simulink model "FullFMS_2026_02_17_V0_3_8"  (R2025b)
settings: Solver=ode23tb  StartTime=0.0  StopTime=inf  MaxStep=0.1  RelTol=1e-2
PreLoadFcn:
  | load("BUS_CONFIG.mat")
libraries: opcualib x8
(part 1 of 4)
settings Model: SimulationMode=accelerator  PacingRate=0.100000  Creator=guilh  LastModifiedBy=vitor
settings SolverCC: ZeroCrossControl=DisableAll

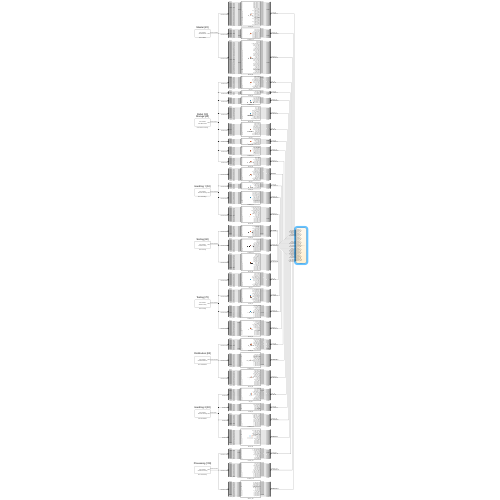
[thumbnail: Simulink's stored preview of the top-level diagram]
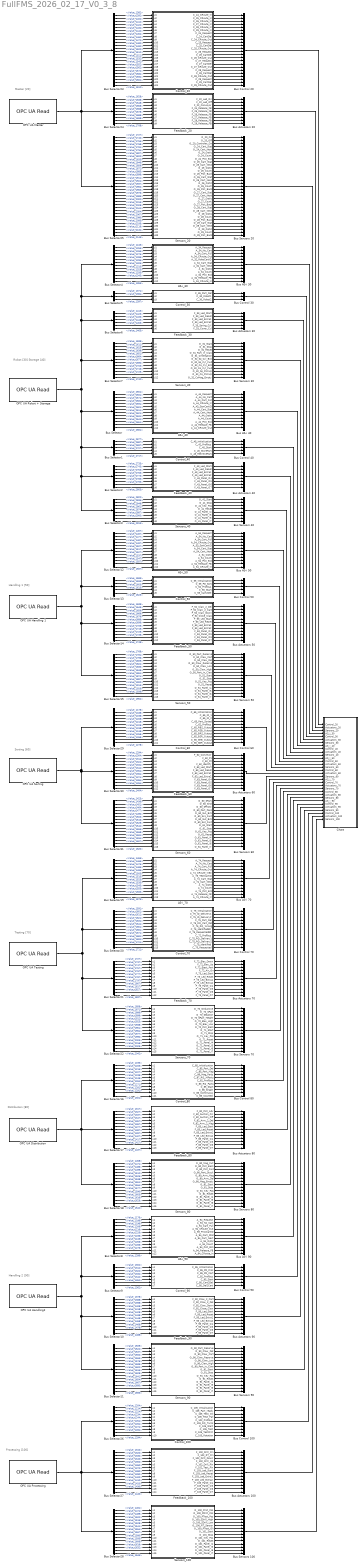
== system FullFMS_2026_02_17_V0_3_8 ==
  note: Master [20]
  note: Robot [30]
      | Storage [40]
  note: Handling 1 [50]
  note: Sorting [60]
  note: Testing [70]
  note: Distribution [80]
  note: Handling 2 [90]
  note: Processing [100]
  AS-i_30 : MATLAB Function  Tag=AS-i  TreatAsAtomicUnit=on
  AS-i_40 : MATLAB Function  TreatAsAtomicUnit=on
  AS-i_50 : MATLAB Function  TreatAsAtomicUnit=on
  AS-i_70 : MATLAB Function  Tag=AS-i  TreatAsAtomicUnit=on
  AS-i_90 : MATLAB Function  Tag=AS-i  TreatAsAtomicUnit=on
  Bus Selector : BusSelector  OutputSignals=Value_2551,Value_2561,Value_2571,Value_2581,Value_2591,Value_2601,Value_2611,Value_2621,Value_2631,Value_2641,Value_2651,Value_2661
  Bus Selector1 : BusSelector  OutputSignals=Value_2677,Value_2687,Value_2697,Value_2707,Value_2717
  Bus Selector10 : BusSelector  OutputSignals=Value_1378,Value_1388,Value_1398,Value_1408,Value_1418,Value_1428,Value_1438,Value_1448,Value_1458,Value_1468,Value_1478,Value_1488
  Bus Selector11 : BusSelector  OutputSignals=Value_1509,Value_1522,Value_1537,Value_1550,Value_1563,Value_1576,Value_1589,Value_1602,Value_1615,Value_1628,Value_1641,Value_1654,Value_1667,Value_1680,Value_1693
  Bus Selector12 : BusSelector  OutputSignals=Value_1457,Value_1467,Value_1477,Value_1487,Value_1497,Value_1507,Value_1517,Value_1527,Value_1537,Value_1547,Value_1557,Value_1567
  Bus Selector13 : BusSelector  OutputSignals=Value_1583,Value_1593,Value_1603,Value_1613,Value_1623
  Bus Selector14 : BusSelector  OutputSignals=Value_1639,Value_1649,Value_1659,Value_1669,Value_1679,Value_1689,Value_1699,Value_1709,Value_1719,Value_1729,Value_1739,Value_1749
  Bus Selector15 : BusSelector  OutputSignals=Value_1768,Value_1781,Value_1796,Value_1809,Value_1822,Value_1835,Value_1848,Value_1861,Value_1874,Value_1887,Value_1900,Value_1913,Value_1926,Value_1939,Value_1952
  Bus Selector16 : BusSelector  OutputSignals=Value_1195,Value_1205,Value_1215,Value_1227,Value_1239,Value_1249,Value_1261,Value_1271,Value_1281,Value_1291,Value_1301
  Bus Selector17 : BusSelector  OutputSignals=Value_1317,Value_1327,Value_1337,Value_1347,Value_1357,Value_1367,Value_1377,Value_1387,Value_1397,Value_1407,Value_1417,Value_1427,Value_1437
  Bus Selector18 : BusSelector  OutputSignals=Value_1458,Value_1471,Value_1486,Value_1499,Value_1512,Value_1525,Value_1538,Value_1551,Value_1564,Value_1577,Value_1590,Value_1603,Value_1616,Value_1629,Value_1642
  Bus Selector19 : BusSelector  OutputSignals=Value_1455,Value_1465,Value_1475,Value_1485,Value_1495,Value_1505,Value_1515,Value_1525,Value_1535,Value_1545,Value_1555,Value_1565,Value_1575
  Bus Selector2 : BusSelector  OutputSignals=Value_2733,Value_2743,Value_2753,Value_2763,Value_2773,Value_2783,Value_2793,Value_2803
  Bus Selector20 : BusSelector  OutputSignals=Value_1591,Value_1601,Value_1611,Value_1621,Value_1631,Value_1641,Value_1651,Value_1661,Value_1671,Value_1681,Value_1691,Value_1701,Value_1711
  Bus Selector21 : BusSelector  OutputSignals=Value_1727,Value_1737,Value_1747,Value_1757,Value_1767,Value_1777,Value_1787,Value_1797,Value_1807,Value_1817,Value_1827,Value_1837
  Bus Selector22 : BusSelector  OutputSignals=Value_1858,Value_1871,Value_1886,Value_1899,Value_1912,Value_1925,Value_1938,Value_1951,Value_1964,Value_1977,Value_1990,Value_2003,Value_2016,Value_2029,Value_2042
  Bus Selector23 : BusSelector  OutputSignals=Value_1382,Value_1392,Value_1402,Value_1412,Value_1422,Value_1432,Value_1442,Value_1452,Value_1462,Value_1472,Value_1482,Value_1492,Value_1502,Value_1512,Value_1522,Value_1532,Value_1542,Value_1552,Value_1562,Value_1572,Value_1582,Value_1592,Value_1602,Value_1612
  Bus Selector24 : BusSelector  OutputSignals=Value_1628,Value_1638,Value_1648,Value_1658,Value_1668,Value_1678,Value_1688,Value_1698,Value_1708
  Bus Selector25 : BusSelector  OutputSignals=Value_1727,Value_1740,Value_1755,Value_1768,Value_1781,Value_1794,Value_1807,Value_1820,Value_1833,Value_1846,Value_1859,Value_1872,Value_1885,Value_1898,Value_1911,Value_1924,Value_1937,Value_1950,Value_1963,Value_1976,Value_1989,Value_2002,Value_2015,Value_2028,Value_2041,Value_2054,Value_2067,Value_2080,Value_2093,Value_2106,Value_2119,Value_2132,Value_2145
  Bus Selector26 : BusSelector  OutputSignals=Value_1204,Value_1214,Value_1224,Value_1234,Value_1244,Value_1254,Value_1264,Value_1274,Value_1284,Value_1294
  Bus Selector27 : BusSelector  OutputSignals=Value_1310,Value_1320,Value_1330,Value_1340,Value_1350,Value_1360,Value_1370,Value_1380,Value_1390,Value_1400,Value_1410,Value_1420,Value_1430,Value_1440
  Bus Selector28 : BusSelector  OutputSignals=Value_1461,Value_1474,Value_1489,Value_1502,Value_1515,Value_1528,Value_1541,Value_1554,Value_1567,Value_1580,Value_1593,Value_1606,Value_1619,Value_1632,Value_1645
  Bus Selector29 : BusSelector  OutputSignals=Value_1178,Value_1188,Value_1198,Value_1208,Value_1218,Value_1228,Value_1238,Value_1248,Value_1258,Value_1268,Value_1278
  Bus Selector3 : BusSelector  OutputSignals=Value_2822,Value_2835,Value_2848,Value_2861,Value_2874,Value_2887,Value_2900,Value_2913
  Bus Selector30 : BusSelector  OutputSignals=Value_1294,Value_1304,Value_1314,Value_1324,Value_1334,Value_1344,Value_1354,Value_1364,Value_1374,Value_1384,Value_1394,Value_1404
  Bus Selector31 : BusSelector  OutputSignals=Value_1423,Value_1436,Value_1451,Value_1464,Value_1477,Value_1490,Value_1503,Value_1516,Value_1529,Value_1542,Value_1555,Value_1568,Value_1581,Value_1594,Value_1607,Value_1620
  Bus Selector4 : BusSelector  OutputSignals=Value_1245,Value_1255,Value_1265,Value_1275,Value_1285,Value_1295,Value_1305,Value_1315,Value_1325,Value_1335,Value_1345,Value_1355
  Bus Selector5 : BusSelector  OutputSignals=Value_1371,Value_1384,Value_1397
  Bus Selector6 : BusSelector  OutputSignals=Value_1413,Value_1423,Value_1433,Value_1443,Value_1453,Value_1463
  Bus Selector7 : BusSelector  OutputSignals=Value_1599,Value_1612,Value_1625,Value_1638,Value_1651,Value_1664,Value_1677,Value_1690,Value_1703,Value_1716,Value_1729,Value_1742
  Bus Selector8 : BusSelector  OutputSignals=Value_1176,Value_1186,Value_1196,Value_1206,Value_1216,Value_1226,Value_1236,Value_1246,Value_1256,Value_1266,Value_1276,Value_1286
  Bus Selector9 : BusSelector  OutputSignals=Value_1302,Value_1312,Value_1322,Value_1332,Value_1342,Value_1352,Value_1362
  Bus AS-i 30 : BusCreator  Inputs=12  OutDataTypeStr=Bus: B_AS_i_30  NonVirtualBus=on
  Bus AS-i 40 : BusCreator  Inputs=12  OutDataTypeStr=Bus: B_AS_i_40  NonVirtualBus=on
  Bus AS-i 50 : BusCreator  Inputs=12  OutDataTypeStr=Bus: B_AS_i_50  NonVirtualBus=on
  Bus AS-i 70 : BusCreator  Inputs=13  OutDataTypeStr=Bus: B_AS_i_70  NonVirtualBus=on
  Bus AS-i 90 : BusCreator  Inputs=12  OutDataTypeStr=Bus: B_AS_i_90  NonVirtualBus=on
  Bus Actuators 100 : BusCreator  Inputs=14  OutDataTypeStr=Bus: B_Actuators_100  NonVirtualBus=on
  Bus Actuators 20 : BusCreator  Inputs=9  OutDataTypeStr=Bus: B_Actuators_20  NonVirtualBus=on
  Bus Actuators 30 : BusCreator  Inputs=6  OutDataTypeStr=Bus: B_Actuators_30  NonVirtualBus=on
  Bus Actuators 40 : BusCreator  Inputs=8  OutDataTypeStr=Bus: B_Actuators_40  NonVirtualBus=on
  Bus Actuators 50 : BusCreator  Inputs=12  OutDataTypeStr=Bus: B_Actuators_50  NonVirtualBus=on
  Bus Actuators 60 : BusCreator  Inputs=12  OutDataTypeStr=Bus: B_Actuators_60  NonVirtualBus=on
  Bus Actuators 70 : BusCreator  Inputs=12  OutDataTypeStr=Bus: B_Actuators_70  NonVirtualBus=on
  Bus Actuators 80 : BusCreator  Inputs=13  OutDataTypeStr=Bus: B_Actuators_80  NonVirtualBus=on
  Bus Actuators 90 : BusCreator  Inputs=12  OutDataTypeStr=Bus: B_Actuators_90  NonVirtualBus=on
  Bus Control 100 : BusCreator  Inputs=10  OutDataTypeStr=Bus: B_Control_100  NonVirtualBus=on
  Bus Control 20 : BusCreator  Inputs=24  OutDataTypeStr=Bus: B_Control_20  NonVirtualBus=on
  Bus Control 30 : BusCreator  Inputs=3  OutDataTypeStr=Bus: B_Control_30  NonVirtualBus=on
  Bus Control 40 : BusCreator  Inputs=5  OutDataTypeStr=Bus: B_Control_40  NonVirtualBus=on
  Bus Control 50 : BusCreator  Inputs=5  OutDataTypeStr=Bus: B_Control_50  NonVirtualBus=on
  Bus Control 60 : BusCreator  Inputs=11  OutDataTypeStr=Bus: B_Control_60  NonVirtualBus=on
  Bus Control 70 : BusCreator  Inputs=13  OutDataTypeStr=Bus: B_Control_70  NonVirtualBus=on
  Bus Control 80 : BusCreator  Inputs=11  OutDataTypeStr=Bus: B_Control_80  NonVirtualBus=on
  Bus Control 90 : BusCreator  Inputs=7  OutDataTypeStr=Bus: B_Control_90  NonVirtualBus=on
  Bus Sensors 100 : BusCreator  Inputs=15  OutDataTypeStr=Bus: B_Sensors_100  NonVirtualBus=on
  Bus Sensors 20 : BusCreator  Inputs=33  OutDataTypeStr=Bus: B_Sensors_20  NonVirtualBus=on
  Bus Sensors 30 : BusCreator  Inputs=12  OutDataTypeStr=Bus: B_Sensors_30  NonVirtualBus=on
  Bus Sensors 40 : BusCreator  Inputs=8  OutDataTypeStr=Bus: B_Sensors_40  NonVirtualBus=on
  Bus Sensors 50 : BusCreator  Inputs=15  OutDataTypeStr=Bus: B_Sensors_50  NonVirtualBus=on
  Bus Sensors 60 : BusCreator  Inputs=16  OutDataTypeStr=Bus: B_Sensors_60  NonVirtualBus=on
  Bus Sensors 70 : BusCreator  Inputs=15  OutDataTypeStr=Bus: B_Sensors_70  NonVirtualBus=on
  Bus Sensors 80 : BusCreator  Inputs=15  OutDataTypeStr=Bus: B_Sensors_80  NonVirtualBus=on
  Bus Sensors 90 : BusCreator  Inputs=15  OutDataTypeStr=Bus: B_Sensors_90  NonVirtualBus=on
  Chart : Stateflow chart  TreatAsAtomicUnit=on
      settings: PortSchema="{\"entries\":[{\"content\":{\"sides\":[{\"content\":{\"connectorIds\":[\"In18\",\"In12\",\"In24\",\"In8\",\"In19\",\"In13\",\"In25\",\"In30\",\"In29\",\"In31\",\"In32\",\"In9\",\"In20\",\"In14\",\"In26\",\"In21\",\"In15\",\"In27\",\"In4\",\"In5\",\"In6\",\"In7\",\"In1\",\"In2\",\"In3\",\"In10\",\"In22\",\"In16\",\"In28\",\"In17\",\"In11\",\"In23\"]},\"type\":\"ConnectorPlacement.EquallySpacedRectSide\",\"uuid\":\"e54bf7d4-7c7d-41d9-a8b8-f479ac319a99\"},{\"content\":{\"side\":\"RIGHT\"},\"type\":\"ConnectorPlacement.EquallySpacedRectSide\",\"uuid\":\"d3c20706-71bd-4e26-b40f-0ee7e71b06ee\"},{\"content\":{\"side\":\"TOP\"},\"type\":\"ConnectorPlacement.EquallySpacedRectSide\",\"uuid\":\"ecfb6920-e95b-4ed8-99f9-df5ce878328e\"}]},\"type\":\"ConnectorPlacement.EquallySpacedConnector\",\"uuid\":\"2e714192-4eea-4e1a-8945-7c827feed48f\"}],\"packageUris\":[\"http://schema.mathworks.com/mf0/Connector/R2020b\"],\"version\":\"1.0\"}"
  Control_100 : MATLAB Function  Tag=Control  TreatAsAtomicUnit=on
  Control_20 : MATLAB Function  Tag=Control  TreatAsAtomicUnit=on
  Control_30 : MATLAB Function  Tag=Control  TreatAsAtomicUnit=on
  Control_40 : MATLAB Function  TreatAsAtomicUnit=on
  Control_50 : MATLAB Function  TreatAsAtomicUnit=on
  Control_60 : MATLAB Function  Tag=Control  TreatAsAtomicUnit=on
  Control_70 : MATLAB Function  Tag=Control  TreatAsAtomicUnit=on
  Control_80 : MATLAB Function  Tag=Control  TreatAsAtomicUnit=on
  Control_90 : MATLAB Function  Tag=Control  TreatAsAtomicUnit=on
  Feedback_100 : MATLAB Function  Tag=Actuators  TreatAsAtomicUnit=on
  Feedback_20 : MATLAB Function  Tag=Actuators  TreatAsAtomicUnit=on
  Feedback_30 : MATLAB Function  Tag=Actuators  TreatAsAtomicUnit=on
  Feedback_40 : MATLAB Function  TreatAsAtomicUnit=on
  Feedback_50 : MATLAB Function  TreatAsAtomicUnit=on
  Feedback_60 : MATLAB Function  Tag=Actuators  TreatAsAtomicUnit=on
  Feedback_70 : MATLAB Function  Tag=Actuators  TreatAsAtomicUnit=on
  Feedback_80 : MATLAB Function  Tag=Actuators  TreatAsAtomicUnit=on
  Feedback_90 : MATLAB Function  Tag=Actuators  TreatAsAtomicUnit=on
  OPC UA Distribution : opcualib/OPC UA Read  SelectedServer=AAS OPC Distribution  ServerList=AAS OPC Distribution  NodeList={ '1', 'Value', '6', '1195', '1'; '2', 'Value', '6', '1205', '1'; '3', 'Value', '6', '1215', '1'; '4', 'Value', '6', '1227', '1'; '5', 'Value', '6', '1239', '1'; '6', 'Value', '6', '1249', '1'; '7', 'Value', '6', '1261', '1'; '8', 'Value', '6', '1271', '1'; '9', 'Value', '6', '1281', '1'; '10', 'Value', '6', '1291', '1'; '11', 'Value', '6', '1301', '1'; '12', 'Value', '6', '1317', '1'; '13', 'Value', '6', '1327', '1'; '14', 'Value', '6', '1337', '1'; '15', 'Value', '6', '1347', '1'; '16', 'Value', '6', '1357', '1'; '17', 'Value', '6', '1367', '1'; '18', 'Value', '6', '1377', '1'; '19', 'Value', '6', '1387', '1'; '20', 'Value', '6', '1397', '1'; '21', 'Value', '6', '1407', '1'; '22', 'Value', '6', '1417', '1'; '23', 'Value', '6', '1427', '1'; '24', 'Value', '6', '1437', '1'; '25', 'Value', '6', '1458', '1'; '26', 'Value', '6', '1471', '1'; '27', 'Value', '6', '1486', '1'; '28', 'Value', '6', '1499', '1'; '29', 'Value', '6', '1512', '1'; '30', 'Value', '6', '1525', '1'; '31', 'Value', '6', '1538', '1'; '32', 'Value', '6', '1551', '1'; '33', 'Value', '6', '1564', '1'; '34', 'Value', '6', '1577', '1'; '35', 'Value', '6', '1590', '1'; '36', 'Value', '6', '1603', '1'; '37', 'Value', '6', '1616', '1'; '38', 'Value', '6', '1629', '1'; '39', 'Value', '6', '1642', '1' }  ShowQualityPort=off  ShowTimestampPort=off  ShowTimestampPortAs=Seconds since start  SampleTime=-1
  OPC UA Handling 1 : opcualib/OPC UA Read  SelectedServer=AAS OPC Handling1  ServerList=AAS OPC Handling1  NodeList={ '1', 'Value', '6', '1457', '1'; '2', 'Value', '6', '1467', '1'; '3', 'Value', '6', '1477', '1'; '4', 'Value', '6', '1487', '1'; '5', 'Value', '6', '1497', '1'; '6', 'Value', '6', '1507', '1'; '7', 'Value', '6', '1517', '1'; '8', 'Value', '6', '1527', '1'; '9', 'Value', '6', '1537', '1'; '10', 'Value', '6', '1547', '1'; '11', 'Value', '6', '1557', '1'; '12', 'Value', '6', '1567', '1'; '13', 'Value', '6', '1583', '1'; '14', 'Value', '6', '1593', '1'; '15', 'Value', '6', '1603', '1'; '16', 'Value', '6', '1613', '1'; '17', 'Value', '6', '1623', '1'; '18', 'Value', '6', '1639', '1'; '19', 'Value', '6', '1649', '1'; '20', 'Value', '6', '1659', '1'; '21', 'Value', '6', '1669', '1'; '22', 'Value', '6', '1679', '1'; '23', 'Value', '6', '1689', '1'; '24', 'Value', '6', '1699', '1'; '25', 'Value', '6', '1709', '1'; '26', 'Value', '6', '1719', '1'; '27', 'Value', '6', '1729', '1'; '28', 'Value', '6', '1739', '1'; '29', 'Value', '6', '1749', '1'; '30', 'Value', '6', '1768', '1'; '31', 'Value', '6', '1781', '1'; '32', 'Value', '6', '1796', '1'; '33', 'Value', '6', '1809', '1'; '34', 'Value', '6', '1822', '1'; '35', 'Value', '6', '1835', '1'; '36', 'Value', '6', '1848', '1'; '37', 'Value', '6', '1861', '1'; '38', 'Value', '6', '1874', '1'; '39', 'Value', '6', '1887', '1'; '40', 'Value', '6', '1900', '1'; '41', 'Value', '6', '1913', '1'; '42', 'Value', '6', '1926', '1'; '43', 'Value', '6', '1939', '1'; '44', 'Value', '6', '1952', '1' }  ShowQualityPort=off  ShowTimestampPort=off  ShowTimestampPortAs=Seconds since start  SampleTime=-1
  OPC UA Handling2 : opcualib/OPC UA Read  SelectedServer=AAS OPC Handling2  ServerList=AAS OPC Handling2  NodeList={ '1', 'Value', '6', '1176', '1'; '2', 'Value', '6', '1186', '1'; '3', 'Value', '6', '1196', '1'; '4', 'Value', '6', '1206', '1'; '5', 'Value', '6', '1216', '1'; '6', 'Value', '6', '1226', '1'; '7', 'Value', '6', '1236', '1'; '8', 'Value', '6', '1246', '1'; '9', 'Value', '6', '1256', '1'; '10', 'Value', '6', '1266', '1'; '11', 'Value', '6', '1276', '1'; '12', 'Value', '6', '1286', '1'; '13', 'Value', '6', '1302', '1'; '14', 'Value', '6', '1312', '1'; '15', 'Value', '6', '1322', '1'; '16', 'Value', '6', '1332', '1'; '17', 'Value', '6', '1342', '1'; '18', 'Value', '6', '1352', '1'; '19', 'Value', '6', '1362', '1'; '20', 'Value', '6', '1378', '1'; '21', 'Value', '6', '1388', '1'; '22', 'Value', '6', '1398', '1'; '23', 'Value', '6', '1408', '1'; '24', 'Value', '6', '1418', '1'; '25', 'Value', '6', '1428', '1'; '26', 'Value', '6', '1438', '1'; '27', 'Value', '6', '1448', '1'; '28', 'Value', '6', '1458', '1'; '29', 'Value', '6', '1468', '1'; '30', 'Value', '6', '1478', '1'; '31', 'Value', '6', '1488', '1'; '32', 'Value', '6', '1509', '1'; '33', 'Value', '6', '1522', '1'; '34', 'Value', '6', '1537', '1'; '35', 'Value', '6', '1550', '1'; '36', 'Value', '6', '1563', '1'; '37', 'Value', '6', '1576', '1'; '38', 'Value', '6', '1589', '1'; '39', 'Value', '6', '1602', '1'; '40', 'Value', '6', '1615', '1'; '41', 'Value', '6', '1628', '1'; '42', 'Value', '6', '1641', '1'; '43', 'Value', '6', '1654', '1'; '44', 'Value', '6', '1667', '1'; '45', 'Value', '6', '1680', '1'; '46', 'Value', '6', '1693', '1' }  ShowQualityPort=off  ShowTimestampPort=off  ShowTimestampPortAs=Seconds since start  SampleTime=-1
  OPC UA Master : opcualib/OPC UA Read  SelectedServer=AAS OPC Master  ServerList=AAS OPC Master  NodeList={ '1', 'Value', '6', '1382', '1'; '2', 'Value', '6', '1392', '1'; '3', 'Value', '6', '1402', '1'; '4', 'Value', '6', '1412', '1'; '5', 'Value', '6', '1422', '1'; '6', 'Value', '6', '1432', '1'; '7', 'Value', '6', '1442', '1'; '8', 'Value', '6', '1452', '1'; '9', 'Value', '6', '1462', '1'; '10', 'Value', '6', '1472', '1'; '11', 'Value', '6', '1482', '1'; '12', 'Value', '6', '1492', '1'; '13', 'Value', '6', '1502', '1'; '14', 'Value', '6', '1512', '1'; '15', 'Value', '6', '1522', '1'; '16', 'Value', '6', '1532', '1'; '17', 'Value', '6', '1542', '1'; '18', 'Value', '6', '1552', '1'; '19', 'Value', '6', '1562', '1'; '20', 'Value', '6', '1572', '1'; '21', 'Value', '6', '1582', '1'; '22', 'Value', '6', '1592', '1'; '23', 'Value', '6', '1602', '1'; '24', 'Value', '6', '1612', '1'; '25', 'Value', '6', '1628', '1'; '26', 'Value', '6', '1638', '1'; '27', 'Value', '6', '1648', '1'; '28', 'Value', '6', '1658', '1'; '29', 'Value', '6', '1668', '1'; '30', 'Value', '6', '1678', '1'; '31', 'Value', '6', '1688', '1'; '32', 'Value', '6', '1698', '1'; '33', 'Value', '6', '1708', '1'; '34', 'Value', '6', '1727', '1'; '35', 'Value', '6', '1740', '1'; '36', 'Value', '6', '1755', '1'; '37', 'Value', '6', '1768', '1'; '38', 'Value', '6', '1781', '1'; '39', 'Value', '6', '1794', '1'; '40', 'Value', '6', '1807', '1'; '41', 'Value', '6', '1820', '1'; '42', 'Value', '6', '1833', '1'; '43', 'Value', '6', '1846', '1'; '44', 'Value', '6', '1859', '1'; '45', 'Value', '6', '1872', '1'; '46', 'Value', '6', '1885', '1'; '47', 'Value', '6', '1898', '1'; '48', 'Value', '6', '1911', '1'; '49', 'Value', '6', '1924', '1'; '50', 'Value', '6', '1937', '1'; '51', 'Value', '6', '1950', '1'; '52', 'Value', '6', '1963', '1'; '53', 'Value', '6', '1976', '1'; '54', 'Value', '6', '1989', '1'; '55', 'Value', '6', '2002', '1'; '56', 'Value', '6', '2015', '1'; '57', 'Value', '6', '2028', '1'; '58', 'Value', '6', '2041', '1'; '59', 'Value', '6', '2054', '1'; '60', 'Value', '6', '2067', '1'; '61', 'Value', '6', '2080', '1'; '62', 'Value', '6', '2093', '1'; '63', 'Value', '6', '2106', '1'; '64', 'Value', '6', '2119', '1'; '65', 'Value', '6', '2132', '1'; '66', 'Value', '6', '2145', '1' }  ShowQualityPort=off  ShowTimestampPort=off  ShowTimestampPortAs=Seconds since start  SampleTime=-1
  OPC UA Processing : opcualib/OPC UA Read  SelectedServer=AAS OPC Processing  ServerList=AAS OPC Processing  NodeList={ '1', 'Value', '6', '1204', '1'; '2', 'Value', '6', '1214', '1'; '3', 'Value', '6', '1224', '1'; '4', 'Value', '6', '1234', '1'; '5', 'Value', '6', '1244', '1'; '6', 'Value', '6', '1254', '1'; '7', 'Value', '6', '1264', '1'; '8', 'Value', '6', '1274', '1'; '9', 'Value', '6', '1284', '1'; '10', 'Value', '6', '1294', '1'; '11', 'Value', '6', '1310', '1'; '12', 'Value', '6', '1320', '1'; '13', 'Value', '6', '1330', '1'; '14', 'Value', '6', '1340', '1'; '15', 'Value', '6', '1350', '1'; '16', 'Value', '6', '1360', '1'; '17', 'Value', '6', '1370', '1'; '18', 'Value', '6', '1380', '1'; '19', 'Value', '6', '1390', '1'; '20', 'Value', '6', '1400', '1'; '21', 'Value', '6', '1410', '1'; '22', 'Value', '6', '1420', '1'; '23', 'Value', '6', '1430', '1'; '24', 'Value', '6', '1440', '1'; '25', 'Value', '6', '1461', '1'; '26', 'Value', '6', '1474', '1'; '27', 'Value', '6', '1489', '1'; '28', 'Value', '6', '1502', '1'; '29', 'Value', '6', '1515', '1'; '30', 'Value', '6', '1528', '1'; '31', 'Value', '6', '1541', '1'; '32', 'Value', '6', '1554', '1'; '33', 'Value', '6', '1567', '1'; '34', 'Value', '6', '1580', '1'; '35', 'Value', '6', '1593', '1'; '36', 'Value', '6', '1606', '1'; '37', 'Value', '6', '1619', '1'; '38', 'Value', '6', '1632', '1'; '39', 'Value', '6', '1645', '1' }  ShowQualityPort=off  ShowTimestampPort=off  ShowTimestampPortAs=Seconds since start  SampleTime=-1
  OPC UA Robot + Storage : opcualib/OPC UA Read  SelectedServer=Node-RED OPCUA  ServerList=Node-RED OPCUA  NodeList={ '1', 'Value', '6', '2551', '1'; '2', 'Value', '6', '2561', '1'; '3', 'Value', '6', '2571', '1'; '4', 'Value', '6', '2581', '1'; '5', 'Value', '6', '2591', '1'; '6', 'Value', '6', '2601', '1'; '7', 'Value', '6', '2611', '1'; '8', 'Value', '6', '2621', '1'; '9', 'Value', '6', '2631', '1'; '10', 'Value', '6', '2641', '1'; '11', 'Value', '6', '2651', '1'; '12', 'Value', '6', '2661', '1'; '13', 'Value', '6', '2677', '1'; '14', 'Value', '6', '2687', '1'; '15', 'Value', '6', '2697', '1'; '16', 'Value', '6', '2707', '1'; '17', 'Value', '6', '2717', '1'; '18', 'Value', '6', '2733', '1'; '19', 'Value', '6', '2743', '1'; '20', 'Value', '6', '2753', '1'; '21', 'Value', '6', '2763', '1'; '22', 'Value', '6', '2773', '1'; '23', 'Value', '6', '2783', '1'; '24', 'Value', '6', '2793', '1'; '25', 'Value', '6', '2803', '1'; '26', 'Value', '6', '2822', '1'; '27', 'Value', '6', '2835', '1'; '28', 'Value', '6', '2848', '1'; '29', 'Value', '6', '2861', '1'; '30', 'Value', '6', '2874', '1'; '31', 'Value', '6', '2887', '1'; '32', 'Value', '6', '2900', '1'; '33', 'Value', '6', '2913', '1'; '34', 'Value', '6', '1245', '1'; '35', 'Value', '6', '1255', '1'; '36', 'Value', '6', '1265', '1'; '37', 'Value', '6', '1275', '1'; '38', 'Value', '6', '1285', '1'; '39', 'Value', '6', '1295', '1'; '40', 'Value', '6', '1305', '1'; '41', 'Value', '6', '1315', '1'; '42', 'Value', '6', '1325', '1'; '43', 'Value', '6', '1335', '1'; '44', 'Value', '6', '1345', '1'; '45', 'Value', '6', '1355', '1'; '46', 'Value', '6', '1371', '1'; '47', 'Value', '6', '1384', '1'; '48', 'Value', '6', '1397', '1'; '49', 'Value', '6', '1413', '1'; '50', 'Value', '6', '1423', '1'; '51', 'Value', '6', '1433', '1'; '52', 'Value', '6', '1443', '1'; '53', 'Value', '6', '1453', '1'; '54', 'Value', '6', '1463', '1'; '55', 'Value', '6', '1599', '1'; '56', 'Value', '6', '1612', '1'; '57', 'Value', '6', '1625', '1'; '58', 'Value', '6', '1638', '1'; '59', 'Value', '6', '1651', '1'; '60', 'Value', '6', '1664', '1'; '61', 'Value', '6', '1677', '1'; '62', 'Value', '6', '1690', '1'; '63', 'Value', '6', '1703', '1'; '64', 'Value', '6', '1716', '1'; '65', 'Value', '6', '1729', '1'; '66', 'Value', '6', '1742', '1' }  ShowQualityPort=off  ShowTimestampPort=off  ShowTimestampPortAs=Seconds since start  SampleTime=-1
  OPC UA Sorting : opcualib/OPC UA Read  SelectedServer=AAS OPC Sorting  ServerList=AAS OPC Sorting  NodeList={ '1', 'Value', '6', '1178', '1'; '2', 'Value', '6', '1188', '1'; '3', 'Value', '6', '1198', '1'; '4', 'Value', '6', '1208', '1'; '5', 'Value', '6', '1218', '1'; '6', 'Value', '6', '1228', '1'; '7', 'Value', '6', '1238', '1'; '8', 'Value', '6', '1248', '1'; '9', 'Value', '6', '1258', '1'; '10', 'Value', '6', '1268', '1'; '11', 'Value', '6', '1278', '1'; '12', 'Value', '6', '1294', '1'; '13', 'Value', '6', '1304', '1'; '14', 'Value', '6', '1314', '1'; '15', 'Value', '6', '1324', '1'; '16', 'Value', '6', '1334', '1'; '17', 'Value', '6', '1344', '1'; '18', 'Value', '6', '1354', '1'; '19', 'Value', '6', '1364', '1'; '20', 'Value', '6', '1374', '1'; '21', 'Value', '6', '1384', '1'; '22', 'Value', '6', '1394', '1'; '23', 'Value', '6', '1404', '1'; '24', 'Value', '6', '1423', '1'; '25', 'Value', '6', '1436', '1'; '26', 'Value', '6', '1451', '1'; '27', 'Value', '6', '1464', '1'; '28', 'Value', '6', '1477', '1'; '29', 'Value', '6', '1490', '1'; '30', 'Value', '6', '1503', '1'; '31', 'Value', '6', '1516', '1'; '32', 'Value', '6', '1529', '1'; '33', 'Value', '6', '1542', '1'; '34', 'Value', '6', '1555', '1'; '35', 'Value', '6', '1568', '1'; '36', 'Value', '6', '1581', '1'; '37', 'Value', '6', '1594', '1'; '38', 'Value', '6', '1607', '1'; '39', 'Value', '6', '1620', '1' }  ShowQualityPort=off  ShowTimestampPort=off  ShowTimestampPortAs=Seconds since start  SampleTime=-1
  OPC UA Testing : opcualib/OPC UA Read  SelectedServer=AAS OPC Testing  ServerList=AAS OPC Testing  NodeList={ '1', 'Value', '6', '1455', '1'; '2', 'Value', '6', '1465', '1'; '3', 'Value', '6', '1475', '1'; '4', 'Value', '6', '1485', '1'; '5', 'Value', '6', '1495', '1'; '6', 'Value', '6', '1505', '1'; '7', 'Value', '6', '1515', '1'; '8', 'Value', '6', '1525', '1'; '9', 'Value', '6', '1535', '1'; '10', 'Value', '6', '1545', '1'; '11', 'Value', '6', '1555', '1'; '12', 'Value', '6', '1565', '1'; '13', 'Value', '6', '1575', '1'; '14', 'Value', '6', '1591', '1'; '15', 'Value', '6', '1601', '1'; '16', 'Value', '6', '1611', '1'; '17', 'Value', '6', '1621', '1'; '18', 'Value', '6', '1631', '1'; '19', 'Value', '6', '1641', '1'; '20', 'Value', '6', '1651', '1'; '21', 'Value', '6', '1661', '1'; '22', 'Value', '6', '1671', '1'; '23', 'Value', '6', '1681', '1'; '24', 'Value', '6', '1691', '1'; '25', 'Value', '6', '1701', '1'; '26', 'Value', '6', '1711', '1'; '27', 'Value', '6', '1727', '1'; '28', 'Value', '6', '1737', '1'; '29', 'Value', '6', '1747', '1'; '30', 'Value', '6', '1757', '1'; '31', 'Value', '6', '1767', '1'; '32', 'Value', '6', '1777', '1'; '33', 'Value', '6', '1787', '1'; '34', 'Value', '6', '1797', '1'; '35', 'Value', '6', '1807', '1'; '36', 'Value', '6', '1817', '1'; '37', 'Value', '6', '1827', '1'; '38', 'Value', '6', '1837', '1'; '39', 'Value', '6', '1858', '1'; '40', 'Value', '6', '1871', '1'; '41', 'Value', '6', '1886', '1'; '42', 'Value', '6', '1899', '1'; '43', 'Value', '6', '1912', '1'; '44', 'Value', '6', '1925', '1'; '45', 'Value', '6', '1938', '1'; '46', 'Value', '6', '1951', '1'; '47', 'Value', '6', '1964', '1'; '48', 'Value', '6', '1977', '1'; '49', 'Value', '6', '1990', '1'; '50', 'Value', '6', '2003', '1'; '51', 'Value', '6', '2016', '1'; '52', 'Value', '6', '2029', '1'; '53', 'Value', '6', '2042', '1' }  ShowQualityPort=off  ShowTimestampPort=off  ShowTimestampPortAs=Seconds since start  SampleTime=-1
  Sensors_100 : MATLAB Function  Tag=Sensors  TreatAsAtomicUnit=on
  Sensors_20 : MATLAB Function  Tag=Sensor  TreatAsAtomicUnit=on
  Sensors_30 : MATLAB Function  Tag=Sensors  TreatAsAtomicUnit=on
  Sensors_40 : MATLAB Function  TreatAsAtomicUnit=on
  Sensors_50 : MATLAB Function  Tag=Sensors  TreatAsAtomicUnit=on
  Sensors_60 : MATLAB Function  Tag=Sensors  TreatAsAtomicUnit=on
  Sensors_70 : MATLAB Function  Tag=Sensors  TreatAsAtomicUnit=on
  Sensors_80 : MATLAB Function  Tag=Sensors  TreatAsAtomicUnit=on
  Sensors_90 : MATLAB Function  Tag=Sensors  TreatAsAtomicUnit=on
  wires:
  Feedback_80/1(F_82_Pist_Adv) -> Bus Actuators 80/1
  Feedback_80/2(F_82_Suction_On) -> Bus Actuators 80/2
  Feedback_80/3(F_82_Suction_Off) -> Bus Actuators 80/3
  Feedback_80/4(F_82_Arm_2_Del) -> Bus Actuators 80/4
  Feedback_80/5(F_82_Arm_2_Mag) -> Bus Actuators 80/5
  Feedback_80/6(F_83_Led_Start) -> Bus Actuators 80/6
  Feedback_80/7(F_83_Led_Reset) -> Bus Actuators 80/7
  Feedback_80/8(F_83_Led_Extra1) -> Bus Actuators 80/8
  Feedback_80/9(F_83_Led_Extra2) -> Bus Actuators 80/9
  Feedback_80/10(F_83_Panel_O4) -> Bus Actuators 80/10
  Feedback_80/11(F_83_Panel_O5) -> Bus Actuators 80/11
  Feedback_80/12(F_83_Panel_O6) -> Bus Actuators 80/12
  Feedback_80/13(F_83_Panel_O7) -> Bus Actuators 80/13
  Sensors_80/1(O_80_Mag_Full) -> Bus Sensors 80/1
  Sensors_80/2(O_80_Pist_Back) -> Bus Sensors 80/2
  Sensors_80/3(O_80_Pist_Fwd) -> Bus Sensors 80/3
  Sensors_80/4(O_80_Part_Stuck) -> Bus Sensors 80/4
  Sensors_80/5(O_80_Arm_Mag) -> Bus Sensors 80/5
  Sensors_80/6(O_80_Arm_Del) -> Bus Sensors 80/6
  Sensors_80/7(O_80_Mag_Empty) -> Bus Sensors 80/7
  Sensors_80/8(O_81_Start) -> Bus Sensors 80/8
  Sensors_80/9(O_81_Stop) -> Bus Sensors 80/9
  Sensors_80/10(O_81_Key_Pos) -> Bus Sensors 80/10
  Sensors_80/11(O_81_Reset) -> Bus Sensors 80/11
  Sensors_80/12(O_81_Panel_I4) -> Bus Sensors 80/12
  Sensors_80/13(O_81_Panel_I5) -> Bus Sensors 80/13
  Sensors_80/14(O_81_Panel_I6) -> Bus Sensors 80/14
  Sensors_80/15(O_81_Panel_I7) -> Bus Sensors 80/15
  AS-i_70/1(A_74_Request) -> Bus AS-i 70/1
  AS-i_70/2(A_74_No_Cart) -> Bus AS-i 70/2
  AS-i_70/3(A_74_Cart_Full) -> Bus AS-i 70/3
  AS-i_70/4(A_74_CRoute_Out) -> Bus AS-i 70/4
  AS-i_70/5(A_74_CRoute_In80) -> Bus AS-i 70/5
  AS-i_70/6(A_73_TestCartID) -> Bus AS-i 70/6
  AS-i_70/7(A_74_Cart_Stat) -> Bus AS-i 70/7
  AS-i_70/8(A_74_Cart_Next) -> Bus AS-i 70/8
  AS-i_70/9(A_74_Optic) -> Bus AS-i 70/9
  AS-i_70/10(A_74_Count) -> Bus AS-i 70/10
  AS-i_70/11(A_74_Pist_Bck) -> Bus AS-i 70/11
  AS-i_70/12(A_74_Release_FB) -> Bus AS-i 70/12
  AS-i_70/13(A_74_CRoute_In) -> Bus AS-i 70/13
  Control_70/1(C_75_Initialization) -> Bus Control 70/1
  Control_70/2(C_75_ID_Delivery1) -> Bus Control 70/2
  Control_70/3(C_75_ID_Delivery2) -> Bus Control 70/3
  Control_70/4(C_75_Part_Del) -> Bus Control 70/4
  Control_70/5(C_75_RQ_Part_Del) -> Bus Control 70/5
  Control_70/6(C_75_RQ_Wrong) -> Bus Control 70/6
  Control_70/7(C_75_Identified80) -> Bus Control 70/7
  Control_70/8(C_75_Requested80) -> Bus Control 70/8
  Control_70/9(C_72_Profibus) -> Bus Control 70/9
  Control_70/10(C_75_RQ_Delivery1) -> Bus Control 70/10
  Control_70/11(C_75_RQ_Delivery2) -> Bus Control 70/11
  Control_70/12(C_75_Identified) -> Bus Control 70/12
  Control_70/13(C_75_Requested) -> Bus Control 70/13
  Feedback_70/1(F_72_Elev_Down) -> Bus Actuators 70/1
  Feedback_70/2(F_72_Elev_Up) -> Bus Actuators 70/2
  Feedback_70/3(F_72_Eject_Part) -> Bus Actuators 70/3
  Feedback_70/4(F_72_Air_On) -> Bus Actuators 70/4
  Feedback_70/5(F_73_Led_Start) -> Bus Actuators 70/5
  Feedback_70/6(F_73_Led_Reset) -> Bus Actuators 70/6
  Feedback_70/7(F_73_Led_Extra1) -> Bus Actuators 70/7
  Feedback_70/8(F_73_Led_Extra2) -> Bus Actuators 70/8
  Feedback_70/9(F_73_Panel_O4) -> Bus Actuators 70/9
  Feedback_70/10(F_73_Panel_O5) -> Bus Actuators 70/10
  Feedback_70/11(F_73_Panel_O6) -> Bus Actuators 70/11
  Feedback_70/12(F_73_Panel_O7) -> Bus Actuators 70/12
  Sensors_70/1(O_70_SInductive) -> Bus Sensors 70/1
  Sensors_70/2(O_70_SPart) -> Bus Sensors 70/2
  Sensors_70/3(O_70_SStation) -> Bus Sensors 70/3
  Sensors_70/4(O_70_SPart_Height) -> Bus Sensors 70/4
  Sensors_70/5(O_70_Elev_High) -> Bus Sensors 70/5
  Sensors_70/6(O_70_Elev_Low) -> Bus Sensors 70/6
  Sensors_70/7(O_70_Pist_Back) -> Bus Sensors 70/7
  Sensors_70/8(O_71_Start) -> Bus Sensors 70/8
  Sensors_70/9(O_71_Stop) -> Bus Sensors 70/9
  Sensors_70/10(O_71_Key_Pos) -> Bus Sensors 70/10
  Sensors_70/11(O_71_Reset) -> Bus Sensors 70/11
  Sensors_70/12(O_71_Panel_I4) -> Bus Sensors 70/12
  Sensors_70/13(O_71_Panel_I5) -> Bus Sensors 70/13
  Sensors_70/14(O_71_Panel_I6) -> Bus Sensors 70/14
  Sensors_70/15(O_71_Panel_I7) -> Bus Sensors 70/15
  Bus Control 80/1 -> Chart/1(Control_80)
  Bus Actuators 80/1 -> Chart/2(Actuators_80)
  Bus Sensors 80/1 -> Chart/3(Sensors_80)
  Bus Sensors 70/1 -> Chart/7(Sensors_70)
  Bus Actuators 70/1 -> Chart/6(Actuators_70)
  Bus Control 70/1 -> Chart/5(Control_70)
  Bus AS-i 70/1 -> Chart/4(AS_i_70)
  Control_20/1(C_24_CRoute_In) -> Bus Control 20/1
  Control_20/2(C_25_CRoute_In) -> Bus Control 20/2
  Control_20/3(C_26_CRoute_In) -> Bus Control 20/3
  Control_20/4(C_27_CRoute_In) -> Bus Control 20/4
  Control_20/5(C_28_CRoute_In) -> Bus Control 20/5
  Control_20/6(C_29_CRoute_In) -> Bus Control 20/6
  Control_20/7(C_24_Request) -> Bus Control 20/7
  Control_20/8(C_24_CartDel) -> Bus Control 20/8
  Control_20/9(C_24_CRoute_Out) -> Bus Control 20/9
  Control_20/10(C_25_Request) -> Bus Control 20/10
  Control_20/11(C_25_CartDel) -> Bus Control 20/11
  Control_20/12(C_25_CRoute_Out) -> Bus Control 20/12
  Control_20/13(C_26_Request) -> Bus Control 20/13
  Control_20/14(C_26_CartDel) -> Bus Control 20/14
  Control_20/15(C_26_CRoute_Out) -> Bus Control 20/15
  Control_20/16(C_27_Request) -> Bus Control 20/16
  Control_20/17(C_27_CartDel) -> Bus Control 20/17
  Control_20/18(C_27_CRoute_Out) -> Bus Control 20/18
  Control_20/19(C_28_Request) -> Bus Control 20/19
  Control_20/20(C_28_CartDel) -> Bus Control 20/20
  Control_20/21(C_28_CRoute_Out) -> Bus Control 20/21
  Control_20/22(C_29_Request) -> Bus Control 20/22
  Control_20/23(C_29_CartDel) -> Bus Control 20/23
  Control_20/24(C_29_CRoute_Out) -> Bus Control 20/24
  Feedback_20/1(F_22_Led_On) -> Bus Actuators 20/1
  Feedback_20/2(F_22_Led_Off) -> Bus Actuators 20/2
  Feedback_20/3(F_22_Conveyor) -> Bus Actuators 20/3
  Feedback_20/4(F_24_Release_FB) -> Bus Actuators 20/4
  Feedback_20/5(F_25_Release_FB) -> Bus Actuators 20/5
  Feedback_20/6(F_26_Release_FB) -> Bus Actuators 20/6
  Feedback_20/7(F_27_Release_FB) -> Bus Actuators 20/7
  Feedback_20/8(F_28_Release_FB) -> Bus Actuators 20/8
  Feedback_20/9(F_29_Release_FB) -> Bus Actuators 20/9
  Sensors_20/1(O_20_On) -> Bus Sensors 20/1
  Sensors_20/2(O_20_Off) -> Bus Sensors 20/2
  Sensors_20/3(O_20_Controler_On) -> Bus Sensors 20/3
  Sensors_20/4(O_24_Cart_Stat) -> Bus Sensors 20/4
  Sensors_20/5(O_24_Cart_Next) -> Bus Sensors 20/5
  Sensors_20/6(O_24_Optic) -> Bus Sensors 20/6
  Sensors_20/7(O_24_Count) -> Bus Sensors 20/7
  Sensors_20/8(O_24_Pist_Bck) -> Bus Sensors 20/8
  Sensors_20/9(O_25_Cart_Stat) -> Bus Sensors 20/9
  Sensors_20/10(O_25_Cart_Next) -> Bus Sensors 20/10
  Sensors_20/11(O_25_Optic) -> Bus Sensors 20/11
  Sensors_20/12(O_25_Count) -> Bus Sensors 20/12
  Sensors_20/13(O_25_Pist_Back) -> Bus Sensors 20/13
  Sensors_20/14(O_26_Cart_Stat) -> Bus Sensors 20/14
  Sensors_20/15(O_26_Cart_Next) -> Bus Sensors 20/15
  Sensors_20/16(O_26_Optic) -> Bus Sensors 20/16
  Sensors_20/17(O_26_Count) -> Bus Sensors 20/17
  Sensors_20/18(O_26_Pist_Back) -> Bus Sensors 20/18
  Sensors_20/19(O_27_Cart_Stat) -> Bus Sensors 20/19
  Sensors_20/20(O_27_Cart_Next) -> Bus Sensors 20/20
  Sensors_20/21(O_27_Optic) -> Bus Sensors 20/21
  Sensors_20/22(O_27_Count) -> Bus Sensors 20/22
  Sensors_20/23(O_27_Pist_Back) -> Bus Sensors 20/23
  Sensors_20/24(O_28_Cart_Stat) -> Bus Sensors 20/24
  Sensors_20/25(O_28_Cart_Next) -> Bus Sensors 20/25
  Sensors_20/26(O_28_Optic) -> Bus Sensors 20/26
  Sensors_20/27(O_28_Count) -> Bus Sensors 20/27
  Sensors_20/28(O_28_Pist_Back) -> Bus Sensors 20/28
  Sensors_20/29(O_29_Cart_Stat) -> Bus Sensors 20/29
  Sensors_20/30(O_29_Cart_Next) -> Bus Sensors 20/30
  Sensors_20/31(O_29_Optic) -> Bus Sensors 20/31
  Sensors_20/32(O_29_Count) -> Bus Sensors 20/32
  Sensors_20/33(O_29_Pist_Back) -> Bus Sensors 20/33
  Bus Control 20/1 -> Chart/18(Control_20)
  Bus Actuators 20/1 -> Chart/12(Actuators_20)
  Bus Sensors 20/1 -> Chart/24(Sensors_20)
  Sensors_50/1(O_50_Part_Reserve) -> Bus Sensors 50/1
  Sensors_50/2(O_50_Claw_Cart) -> Bus Sensors 50/2
  Sensors_50/3(O_50_Claw_Del) -> Bus Sensors 50/3
  Sensors_50/4(O_50_Claw_Reserve) -> Bus Sensors 50/4
  Sensors_50/5(O_50_Claw_Low) -> Bus Sensors 50/5
  Sensors_50/6(O_50_Claw_High) -> Bus Sensors 50/6
  Sensors_50/7(O_50_Part_in_Claw) -> Bus Sensors 50/7
  Sensors_50/8(O_51_Start) -> Bus Sensors 50/8
  Sensors_50/9(O_51_Stop) -> Bus Sensors 50/9
  Sensors_50/10(O_51_Key_Pos) -> Bus Sensors 50/10
  Sensors_50/11(O_51_Reset) -> Bus Sensors 50/11
  Sensors_50/12(O_51_Panel_I4) -> Bus Sensors 50/12
  Sensors_50/13(O_51_Panel_I5) -> Bus Sensors 50/13
  Sensors_50/14(O_51_Panel_I6) -> Bus Sensors 50/14
  Sensors_50/15(O_51_Panel_I7) -> Bus Sensors 50/15
  Feedback_50/1(F_52_Claw_2_Del) -> Bus Actuators 50/1
  Feedback_50/2(F_52_Claw_2_Cart) -> Bus Actuators 50/2
  Feedback_50/3(F_52_Claw_Down) -> Bus Actuators 50/3
  Feedback_50/4(F_52_Close_Claw) -> Bus Actuators 50/4
  Feedback_50/5(F_53_Led_Start) -> Bus Actuators 50/5
  Feedback_50/6(F_53_Led_Reset) -> Bus Actuators 50/6
  Feedback_50/7(F_53_Led_Extra1) -> Bus Actuators 50/7
  Feedback_50/8(F_53_Led_Extra2) -> Bus Actuators 50/8
  Feedback_50/9(F_53_Panel_O4) -> Bus Actuators 50/9
  Feedback_50/10(F_53_Panel_O5) -> Bus Actuators 50/10
  Feedback_50/11(F_53_Panel_O6) -> Bus Actuators 50/11
  Feedback_50/12(F_53_Panel_O7) -> Bus Actuators 50/12
  Control_50/1(C_55_Initialization) -> Bus Control 50/1
  Control_50/2(C_55_PD_Sort) -> Bus Control 50/2
  Control_50/3(C_52_Profibus) -> Bus Control 50/3
  Control_50/4(C_55_Start) -> Bus Control 50/4
  Control_50/5(C_55_Cart2Del) -> Bus Control 50/5
  Bus AS-i 50/1 -> Chart/9(AS_i_50)
  Bus Control 50/1 -> Chart/20(Control_50)
  Bus Actuators 50/1 -> Chart/14(Actuators_50)
  Bus Sensors 50/1 -> Chart/26(Sensors_50)
  AS-i_90/1(A_94_Request) -> Bus AS-i 90/1
  AS-i_90/2(A_94_No_Cart) -> Bus AS-i 90/2
  AS-i_90/3(A_94_Cart_Full) -> Bus AS-i 90/3
  AS-i_90/4(A_94_CRoute_Out) -> Bus AS-i 90/4
  AS-i_90/5(A_93_ProcCartID) -> Bus AS-i 90/5
  AS-i_90/6(A_94_Cart_Stat) -> Bus AS-i 90/6
  AS-i_90/7(A_94_Cart_Next) -> Bus AS-i 90/7
  AS-i_90/8(A_94_Optic) -> Bus AS-i 90/8
  AS-i_90/9(A_94_Count) -> Bus AS-i 90/9
  AS-i_90/10(A_94_Pist_Bck) -> Bus AS-i 90/10
  AS-i_90/11(A_94_Release_FB) -> Bus AS-i 90/11
  AS-i_90/12(A_94_CRoute_In) -> Bus AS-i 90/12
  Control_90/1(C_95_Initialization) -> Bus Control 90/1
  Control_90/2(C_95_PD_Proc) -> Bus Control 90/2
  Control_90/3(C_95_PD_Cart) -> Bus Control 90/3
  Control_90/4(C_92_Profibus) -> Bus Control 90/4
  Control_90/5(C_95_Start) -> Bus Control 90/5
  Control_90/6(C_95_Cart2Del) -> Bus Control 90/6
  Control_90/7(C_95_Del2Cart) -> Bus Control 90/7
  Feedback_90/1(F_92_Claw_2_Cart) -> Bus Actuators 90/1
  Feedback_90/2(F_92_Claw_2_Del) -> Bus Actuators 90/2
  Feedback_90/3(F_92_Claw_Down) -> Bus Actuators 90/3
  Feedback_90/4(F_92_Close_Claw) -> Bus Actuators 90/4
  Feedback_90/5(F_93_Led_Start) -> Bus Actuators 90/5
  Feedback_90/6(F_93_Led_Reset) -> Bus Actuators 90/6
  Feedback_90/7(F_93_Led_Extra1) -> Bus Actuators 90/7
  Feedback_90/8(F_93_Led_Extra2) -> Bus Actuators 90/8
  Feedback_90/9(F_93_Panel_O4) -> Bus Actuators 90/9
  Feedback_90/10(F_93_Panel_O5) -> Bus Actuators 90/10
  Feedback_90/11(F_93_Panel_O6) -> Bus Actuators 90/11
  Feedback_90/12(F_93_Panel_O7) -> Bus Actuators 90/12
  Sensors_90/1(O_90_Part_Reserve) -> Bus Sensors 90/1
  Sensors_90/2(O_90_Claw_Del) -> Bus Sensors 90/2
  Sensors_90/3(O_90_Claw_Cart) -> Bus Sensors 90/3
  Sensors_90/4(O_90_Claw_Reserve) -> Bus Sensors 90/4
  Sensors_90/5(O_90_Claw_Low) -> Bus Sensors 90/5
  Sensors_90/6(O_90_Claw_High) -> Bus Sensors 90/6
  Sensors_90/7(O_90_Part_in_Claw) -> Bus Sensors 90/7
  Sensors_90/8(O_91_Start) -> Bus Sensors 90/8
  Sensors_90/9(O_91_Stop) -> Bus Sensors 90/9
  Sensors_90/10(O_91_Key_Pos) -> Bus Sensors 90/10
  Sensors_90/11(O_91_Reset) -> Bus Sensors 90/11
  Sensors_90/12(O_91_Panel_I4) -> Bus Sensors 90/12
  Sensors_90/13(O_91_Panel_I5) -> Bus Sensors 90/13
  Sensors_90/14(O_91_Panel_I6) -> Bus Sensors 90/14
  Sensors_90/15(O_91_Panel_I7) -> Bus Sensors 90/15
  Bus AS-i 90/1 -> Chart/10(AS_i_90)
  Bus Control 90/1 -> Chart/22(Control_90)
  Bus Actuators 90/1 -> Chart/16(Actuators_90)
  Bus Sensors 90/1 -> Chart/28(Sensors_90)
  Sensors_100/1(O_100_PInit_Pos) -> Bus Sensors 100/1
  Sensors_100/2(O_100_PDrill_Pos) -> Bus Sensors 100/2
  Sensors_100/3(O_100_PTest_Pos) -> Bus Sensors 100/3
  Sensors_100/4(O_100_SDrill_High) -> Bus Sensors 100/4
  Sensors_100/5(O_100_SDrill_Low) -> Bus Sensors 100/5
  Sensors_100/6(O_100_RT_Sensor) -> Bus Sensors 100/6
  Sensors_100/7(O_100_PTest_Ok) -> Bus Sensors 100/7
  Sensors_100/8(O_101_Start) -> Bus Sensors 100/8
  Sensors_100/9(O_101_Stop) -> Bus Sensors 100/9
  Sensors_100/10(O_101_Key_Pos) -> Bus Sensors 100/10
  Sensors_100/11(O_101_Reset) -> Bus Sensors 100/11
  Sensors_100/12(O_101_Panel_I4) -> Bus Sensors 100/12
  Sensors_100/13(O_101_Panel_I5) -> Bus Sensors 100/13
  Sensors_100/14(O_101_Panel_I6) -> Bus Sensors 100/14
  Sensors_100/15(O_101_Panel_I7) -> Bus Sensors 100/15
  Control_100/1(C_105_Initialization) -> Bus Control 100/1
  Control_100/2(C_105_Part_ready) -> Bus Control 100/2
  Control_100/3(C_105_Test_Ok) -> Bus Control 100/3
  Control_100/4(C_105_Test_Fail) -> Bus Control 100/4
  Control_100/5(C_102_Profibus) -> Bus Control 100/5
  Control_100/6(C_103_RQ_Turns) -> Bus Control 100/6
  Control_100/7(C_105_Start) -> Bus Control 100/7
  Control_100/8(C_105_Test) -> Bus Control 100/8
  Control_100/9(C_105_TestDrill) -> Bus Control 100/9
  Control_100/10(C_105_Rotation) -> Bus Control 100/10
  Feedback_100/1(F_102_Drill_On) -> Bus Actuators 100/1
  Feedback_100/2(F_102_RT_On) -> Bus Actuators 100/2
  Feedback_100/3(F_102_Drill_Down) -> Bus Actuators 100/3
  Feedback_100/4(F_102_Drill_Up) -> Bus Actuators 100/4
  Feedback_100/5(F_102_Drill_Pin) -> Bus Actuators 100/5
  Feedback_100/6(F_102_Test_Pin) -> Bus Actuators 100/6
  Feedback_100/7(F_103_Led_Start) -> Bus Actuators 100/7
  Feedback_100/8(F_103_Led_Reset) -> Bus Actuators 100/8
  Feedback_100/9(F_103_Led_Extra1) -> Bus Actuators 100/9
  Feedback_100/10(F_103_Led_Extra2) -> Bus Actuators 100/10
  Feedback_100/11(F_103_Panel_O4) -> Bus Actuators 100/11
  Feedback_100/12(F_103_Panel_O5) -> Bus Actuators 100/12
  Feedback_100/13(F_103_Panel_O6) -> Bus Actuators 100/13
  Feedback_100/14(F_103_Panel_O7) -> Bus Actuators 100/14
  Bus Control 100/1 -> Chart/17(Control_100)
  Bus Actuators 100/1 -> Chart/11(Actuators_100)
  Bus Sensors 100/1 -> Chart/23(Sensors_100)
  AS-i_30/1(A_34_Request) -> Bus AS-i 30/1
  AS-i_30/2(A_34_No_Cart) -> Bus AS-i 30/2
  AS-i_30/3(A_34_Cart_Full) -> Bus AS-i 30/3
  AS-i_30/4(A_34_CRoute_Out) -> Bus AS-i 30/4
  AS-i_30/5(A_32_RoboCartID) -> Bus AS-i 30/5
  AS-i_30/6(A_34_Cart_Stat) -> Bus AS-i 30/6
  AS-i_30/7(A_34_Cart_Next) -> Bus AS-i 30/7
  AS-i_30/8(A_34_Optic) -> Bus AS-i 30/8
  AS-i_30/9(A_34_Count) -> Bus AS-i 30/9
  AS-i_30/10(A_34_Pist_Bck) -> Bus AS-i 30/10
  AS-i_30/11(A_34_Release_FB) -> Bus AS-i 30/11
  AS-i_30/12(A_34_CRoute_In) -> Bus AS-i 30/12
  Feedback_30/1(F_33_Led_Start) -> Bus Actuators 30/1
  Feedback_30/2(F_33_Led_Reset) -> Bus Actuators 30/2
  Feedback_30/3(F_33_Led_Extra1) -> Bus Actuators 30/3
  Feedback_30/4(F_33_Led_Extra2) -> Bus Actuators 30/4
  Feedback_30/5(F_33_Spring_Cyl) -> Bus Actuators 30/5
  Feedback_30/6(F_33_Cover_Cyl) -> Bus Actuators 30/6
  Sensors_30/1(O_31_Start) -> Bus Sensors 30/1
  Sensors_30/2(O_31_Stop) -> Bus Sensors 30/2
  Sensors_30/3(O_31_Reset) -> Bus Sensors 30/3
  Sensors_30/4(O_31_Part_in_Claw) -> Bus Sensors 30/4
  Sensors_30/5(O_31_Orientation) -> Bus Sensors 30/5
  Sensors_30/6(O_32_Sp_Cyl_Bck) -> Bus Sensors 30/6
  Sensors_30/7(O_32_Sp_Cyl_Fwd) -> Bus Sensors 30/7
  Sensors_30/8(O_32_Co_Cyl_Bck) -> Bus Sensors 30/8
  Sensors_30/9(O_32_Co_Cyl_Fwd) -> Bus Sensors 30/9
  Sensors_30/10(O_32_Sp_PickUp) -> Bus Sensors 30/10
  Sensors_30/11(O_32_Co_PickUp) -> Bus Sensors 30/11
  Sensors_30/12(O_32_CoMag_Empty) -> Bus Sensors 30/12
  Bus AS-i 30/1 -> Chart/8(AS_i_30)
  Bus Control 30/1 -> Chart/19(Control_30)
  Bus Actuators 30/1 -> Chart/13(Actuators_30)
  Bus Sensors 30/1 -> Chart/25(Sensors_30)
  Control_60/1(C_65_Initialization) -> Bus Control 60/1
  Control_60/2(C_65_ID_1) -> Bus Control 60/2
  Control_60/3(C_65_ID_2) -> Bus Control 60/3
  Control_60/4(C_65_Part_Sorted) -> Bus Control 60/4
  Control_60/5(C_62_Profibus) -> Bus Control 60/5
  Control_60/6(C_65_RBS_Output) -> Bus Control 60/6
  Control_60/7(C_65_RSB_Output) -> Bus Control 60/7
  Control_60/8(C_65_BRS_Output) -> Bus Control 60/8
  Control_60/9(C_65_BSR_Output) -> Bus Control 60/9
  Control_60/10(C_65_SRB_Output) -> Bus Control 60/10
  Control_60/11(C_65_SBR_Output) -> Bus Control 60/11
  Feedback_60/1(F_62_Conveyor) -> Bus Actuators 60/1
  Feedback_60/2(F_62_P1) -> Bus Actuators 60/2
  Feedback_60/3(F_62_P2) -> Bus Actuators 60/3
  Feedback_60/4(F_62_Identify) -> Bus Actuators 60/4
  Feedback_60/5(F_63_Led_Start) -> Bus Actuators 60/5
  Feedback_60/6(F_63_Led_Reset) -> Bus Actuators 60/6
  Feedback_60/7(F_63_Led_Extra1) -> Bus Actuators 60/7
  Feedback_60/8(F_63_Led_Extra2) -> Bus Actuators 60/8
  Feedback_60/9(F_63_Panel_O4) -> Bus Actuators 60/9
  Feedback_60/10(F_63_Panel_O5) -> Bus Actuators 60/10
  Feedback_60/11(F_63_Panel_O6) -> Bus Actuators 60/11
  Feedback_60/12(F_63_Panel_O7) -> Bus Actuators 60/12
  Sensors_60/1(O_60_SPart) -> Bus Sensors 60/1
  Sensors_60/2(O_60_Slnd) -> Bus Sensors 60/2
  Sensors_60/3(O_60_SPhoto) -> Bus Sensors 60/3
  Sensors_60/4(O_60_Part_Pass) -> Bus Sensors 60/4
  Sensors_60/5(O_60_SL1_Bck) -> Bus Sensors 60/5
  Sensors_60/6(O_60_SL1_Fwd) -> Bus Sensors 60/6
  Sensors_60/7(O_60_SL2_Bck) -> Bus Sensors 60/7
  Sensors_60/8(O_60_SL2_Fwd) -> Bus Sensors 60/8
  Sensors_60/9(O_61_Start) -> Bus Sensors 60/9
  Sensors_60/10(O_61_Stop) -> Bus Sensors 60/10
  Sensors_60/11(O_61_Key_Pos) -> Bus Sensors 60/11
  Sensors_60/12(O_61_Reset) -> Bus Sensors 60/12
  Sensors_60/13(O_61_Panel_I4) -> Bus Sensors 60/13
  Sensors_60/14(O_61_Panel_I5) -> Bus Sensors 60/14
  Sensors_60/15(O_61_Panel_I6) -> Bus Sensors 60/15
  Sensors_60/16(O_61_Panel_I7) -> Bus Sensors 60/16
  Bus Control 60/1 -> Chart/21(Control_60)
  Bus Actuators 60/1 -> Chart/15(Actuators_60)
  Bus Sensors 60/1 -> Chart/27(Sensors_60)
  Control_40/1(C_45_Initialization) -> Bus Control 40/1
  Control_40/2(C_42_Profibus) -> Bus Control 40/2
  Control_40/3(C_45_Start) -> Bus Control 40/3
  Control_40/4(C_45_StorePart) -> Bus Control 40/4
  Control_40/5(C_45_RetrievePart) -> Bus Control 40/5
  Feedback_40/1(F_43_Led_Start) -> Bus Actuators 40/1
  Feedback_40/2(F_43_Led_Reset) -> Bus Actuators 40/2
  Feedback_40/3(F_43_Led_Extra1) -> Bus Actuators 40/3
  Feedback_40/4(F_43_Led_Extra2) -> Bus Actuators 40/4
  Feedback_40/5(F_43_Panel_O4) -> Bus Actuators 40/5
  Feedback_40/6(F_43_Panel_O5) -> Bus Actuators 40/6
  Feedback_40/7(F_43_Panel_O6) -> Bus Actuators 40/7
  Feedback_40/8(F_43_Panel_O7) -> Bus Actuators 40/8
  Sensors_40/1(O_41_Start) -> Bus Sensors 40/1
  Sensors_40/2(O_41_Stop) -> Bus Sensors 40/2
  Sensors_40/3(O_41_Key_Pos) -> Bus Sensors 40/3
  Sensors_40/4(O_41_Reset) -> Bus Sensors 40/4
  Sensors_40/5(O_41_Panel_I4) -> Bus Sensors 40/5
  Sensors_40/6(O_41_Panel_I5) -> Bus Sensors 40/6
  Sensors_40/7(O_41_Panel_I6) -> Bus Sensors 40/7
  Sensors_40/8(O_41_Panel_I7) -> Bus Sensors 40/8
  Bus AS-i 40/1 -> Chart/30(AS_i_40)
  Bus Control 40/1 -> Chart/29(Control_40)
  Bus Actuators 40/1 -> Chart/31(Actuators_40)
  Bus Sensors 40/1 -> Chart/32(Sensors_40)
  Control_80/1(C_85_Initialization) -> Bus Control 80/1
  Control_80/2(C_85_Part_Del) -> Bus Control 80/2
  Control_80/3(C_85_Part_Mag) -> Bus Control 80/3
  Control_80/4(C_86_Mag_Parts) -> Bus Control 80/4
  Control_80/5(C_87_RQ_MParts) -> Bus Control 80/5
  Control_80/6(C_82_Profibus) -> Bus Control 80/6
  Control_80/7(C_83_RQ_Parts) -> Bus Control 80/7
  Control_80/8(C_85_Start) -> Bus Control 80/8
  Control_80/9(C_85_Single) -> Bus Control 80/9
  Control_80/10(C_85_Continuous) -> Bus Control 80/10
  Control_80/11(C_85_Counted) -> Bus Control 80/11
  AS-i_50/1(A_54_Request) -> Bus AS-i 50/1
  AS-i_50/2(A_54_No_Cart) -> Bus AS-i 50/2
  AS-i_50/3(A_54_Cart_Full) -> Bus AS-i 50/3
  AS-i_50/4(A_54_CRoute_Out) -> Bus AS-i 50/4
  AS-i_50/5(A_53_SortCartID) -> Bus AS-i 50/5
  AS-i_50/6(A_54_Cart_Stat) -> Bus AS-i 50/6
  AS-i_50/7(A_54_Cart_Next) -> Bus AS-i 50/7
  AS-i_50/8(A_54_Optic) -> Bus AS-i 50/8
  AS-i_50/9(A_54_Count) -> Bus AS-i 50/9
  AS-i_50/10(A_54_Pist_Bck) -> Bus AS-i 50/10
  AS-i_50/11(A_54_Release_FB) -> Bus AS-i 50/11
  AS-i_50/12(A_54_CRoute_In) -> Bus AS-i 50/12
  Control_30/1(C_35_Part_Del) -> Bus Control 30/1
  Control_30/2(C_30_Robot1) -> Bus Control 30/2
  Control_30/3(C_30_Robot2) -> Bus Control 30/3
  AS-i_40/1(A_44_Request) -> Bus AS-i 40/1
  AS-i_40/2(A_44_No_Cart) -> Bus AS-i 40/2
  AS-i_40/3(A_44_Cart_Full) -> Bus AS-i 40/3
  AS-i_40/4(A_44_CRoute_In) -> Bus AS-i 40/4
  AS-i_40/5(A_43_StorCartID) -> Bus AS-i 40/5
  AS-i_40/6(A_44_Cart_Stat) -> Bus AS-i 40/6
  AS-i_40/7(A_44_Cart_Next) -> Bus AS-i 40/7
  AS-i_40/8(A_44_Optic) -> Bus AS-i 40/8
  AS-i_40/9(A_44_Count) -> Bus AS-i 40/9
  AS-i_40/10(A_44_Pist_Bck) -> Bus AS-i 40/10
  AS-i_40/11(A_44_Release_FB) -> Bus AS-i 40/11
  AS-i_40/12(A_44_CRoute_Out) -> Bus AS-i 40/12
  Bus Selector/1 -> AS-i_40/1(u1)  "<Value_2551>"
  Bus Selector/2 -> AS-i_40/2(u2)  "<Value_2561>"
  Bus Selector/3 -> AS-i_40/3(u3)  "<Value_2571>"
  Bus Selector/4 -> AS-i_40/4(u4)  "<Value_2581>"
  Bus Selector/5 -> AS-i_40/5(u5)  "<Value_2591>"
  Bus Selector/6 -> AS-i_40/6(u6)  "<Value_2601>"
  Bus Selector/7 -> AS-i_40/7(u7)  "<Value_2611>"
  Bus Selector/8 -> AS-i_40/8(u8)  "<Value_2621>"
  Bus Selector/9 -> AS-i_40/9(u9)  "<Value_2631>"
  Bus Selector/10 -> AS-i_40/10(u10)  "<Value_2641>"
  Bus Selector/11 -> AS-i_40/11(u11)  "<Value_2651>"
  Bus Selector/12 -> AS-i_40/12(u12)  "<Value_2661>"
  Bus Selector1/1 -> Control_40/1(u1)  "<Value_2677>"
  Bus Selector1/2 -> Control_40/2(u2)  "<Value_2687>"
  Bus Selector1/3 -> Control_40/3(u3)  "<Value_2697>"
  Bus Selector1/4 -> Control_40/4(u4)  "<Value_2707>"
  Bus Selector1/5 -> Control_40/5(u5)  "<Value_2717>"
  Bus Selector2/1 -> Feedback_40/1(u1)  "<Value_2733>"
  Bus Selector2/2 -> Feedback_40/2(u2)  "<Value_2743>"
  Bus Selector2/3 -> Feedback_40/3(u3)  "<Value_2753>"
  Bus Selector2/4 -> Feedback_40/4(u4)  "<Value_2763>"
  Bus Selector2/5 -> Feedback_40/5(u5)  "<Value_2773>"
  Bus Selector2/6 -> Feedback_40/6(u6)  "<Value_2783>"
  Bus Selector2/7 -> Feedback_40/7(u7)  "<Value_2793>"
  Bus Selector2/8 -> Feedback_40/8(u8)  "<Value_2803>"
  Bus Selector3/1 -> Sensors_40/1(u1)  "<Value_2822>"
  Bus Selector3/2 -> Sensors_40/2(u2)  "<Value_2835>"
  Bus Selector3/3 -> Sensors_40/3(u3)  "<Value_2848>"
  Bus Selector3/4 -> Sensors_40/4(u4)  "<Value_2861>"
  Bus Selector3/5 -> Sensors_40/5(u5)  "<Value_2874>"
  Bus Selector3/6 -> Sensors_40/6(u6)  "<Value_2887>"
  Bus Selector3/7 -> Sensors_40/7(u7)  "<Value_2900>"
  Bus Selector3/8 -> Sensors_40/8(u8)  "<Value_2913>"
  Bus Selector4/1 -> AS-i_30/1(u1)  "<Value_1245>"
  Bus Selector4/2 -> AS-i_30/2(u2)  "<Value_1255>"
  Bus Selector4/3 -> AS-i_30/3(u3)  "<Value_1265>"
  Bus Selector4/4 -> AS-i_30/4(u4)  "<Value_1275>"
  Bus Selector4/5 -> AS-i_30/5(u5)  "<Value_1285>"
  Bus Selector4/6 -> AS-i_30/6(u6)  "<Value_1295>"
  Bus Selector4/7 -> AS-i_30/7(u7)  "<Value_1305>"
  Bus Selector4/8 -> AS-i_30/8(u8)  "<Value_1315>"
  Bus Selector4/9 -> AS-i_30/9(u9)  "<Value_1325>"
  Bus Selector4/10 -> AS-i_30/10(u10)  "<Value_1335>"
  Bus Selector4/11 -> AS-i_30/11(u11)  "<Value_1345>"
  Bus Selector4/12 -> AS-i_30/12(u12)  "<Value_1355>"
  Bus Selector5/1 -> Control_30/1(u1)  "<Value_1371>"
  Bus Selector5/2 -> Control_30/2(u2)  "<Value_1384>"
  Bus Selector5/3 -> Control_30/3(u3)  "<Value_1397>"
  Bus Selector6/1 -> Feedback_30/1(u1)  "<Value_1413>"
  Bus Selector6/2 -> Feedback_30/2(u2)  "<Value_1423>"
  Bus Selector6/3 -> Feedback_30/3(u3)  "<Value_1433>"
  Bus Selector6/4 -> Feedback_30/4(u4)  "<Value_1443>"
  Bus Selector6/5 -> Feedback_30/5(u5)  "<Value_1453>"
  Bus Selector6/6 -> Feedback_30/6(u6)  "<Value_1463>"
  Bus Selector7/1 -> Sensors_30/1(u1)  "<Value_1599>"
  Bus Selector7/2 -> Sensors_30/2(u2)  "<Value_1612>"
  Bus Selector7/3 -> Sensors_30/3(u3)  "<Value_1625>"
  Bus Selector7/4 -> Sensors_30/4(u4)  "<Value_1638>"
  Bus Selector7/5 -> Sensors_30/5(u5)  "<Value_1651>"
  Bus Selector7/6 -> Sensors_30/6(u6)  "<Value_1664>"
  Bus Selector7/7 -> Sensors_30/7(u7)  "<Value_1677>"
  Bus Selector7/8 -> Sensors_30/8(u8)  "<Value_1690>"
  Bus Selector7/9 -> Sensors_30/9(u9)  "<Value_1703>"
  Bus Selector7/10 -> Sensors_30/10(u10)  "<Value_1716>"
  Bus Selector7/11 -> Sensors_30/11(u11)  "<Value_1729>"
  Bus Selector7/12 -> Sensors_30/12(u12)  "<Value_1742>"
  OPC UA Handling2/1 -> Bus Selector10/1, Bus Selector11/1, Bus Selector8/1, Bus Selector9/1
  Bus Selector8/1 -> AS-i_90/1(u1)  "<Value_1176>"
  Bus Selector8/2 -> AS-i_90/2(u2)  "<Value_1186>"
  Bus Selector8/3 -> AS-i_90/3(u3)  "<Value_1196>"
  Bus Selector8/4 -> AS-i_90/4(u4)  "<Value_1206>"
  Bus Selector8/5 -> AS-i_90/5(u5)  "<Value_1216>"
  Bus Selector8/6 -> AS-i_90/6(u6)  "<Value_1226>"
  Bus Selector8/7 -> AS-i_90/7(u7)  "<Value_1236>"
  Bus Selector8/8 -> AS-i_90/8(u8)  "<Value_1246>"
  Bus Selector8/9 -> AS-i_90/9(u9)  "<Value_1256>"
  Bus Selector8/10 -> AS-i_90/10(u10)  "<Value_1266>"
  Bus Selector8/11 -> AS-i_90/11(u11)  "<Value_1276>"
  Bus Selector8/12 -> AS-i_90/12(u12)  "<Value_1286>"
  Bus Selector9/1 -> Control_90/1(u1)  "<Value_1302>"
  Bus Selector9/2 -> Control_90/2(u2)  "<Value_1312>"
  Bus Selector9/3 -> Control_90/3(u3)  "<Value_1322>"
  Bus Selector9/4 -> Control_90/4(u4)  "<Value_1332>"
  Bus Selector9/5 -> Control_90/5(u5)  "<Value_1342>"
  Bus Selector9/6 -> Control_90/6(u6)  "<Value_1352>"
  Bus Selector9/7 -> Control_90/7(u7)  "<Value_1362>"
  Bus Selector10/1 -> Feedback_90/1(u1)  "<Value_1378>"
  Bus Selector10/2 -> Feedback_90/2(u2)  "<Value_1388>"
  Bus Selector10/3 -> Feedback_90/3(u3)  "<Value_1398>"
  Bus Selector10/4 -> Feedback_90/4(u4)  "<Value_1408>"
  Bus Selector10/5 -> Feedback_90/5(u5)  "<Value_1418>"
  Bus Selector10/6 -> Feedback_90/6(u6)  "<Value_1428>"
  Bus Selector10/7 -> Feedback_90/7(u7)  "<Value_1438>"
  Bus Selector10/8 -> Feedback_90/8(u8)  "<Value_1448>"
  Bus Selector10/9 -> Feedback_90/9(u9)  "<Value_1458>"
  Bus Selector10/10 -> Feedback_90/10(u10)  "<Value_1468>"
  Bus Selector10/11 -> Feedback_90/11(u11)  "<Value_1478>"
  Bus Selector10/12 -> Feedback_90/12(u12)  "<Value_1488>"
  Bus Selector11/1 -> Sensors_90/1(u1)  "<Value_1509>"
  Bus Selector11/2 -> Sensors_90/2(u2)  "<Value_1522>"
  Bus Selector11/3 -> Sensors_90/3(u3)  "<Value_1537>"
  Bus Selector11/4 -> Sensors_90/4(u4)  "<Value_1550>"
  Bus Selector11/5 -> Sensors_90/5(u5)  "<Value_1563>"
  Bus Selector11/6 -> Sensors_90/6(u6)  "<Value_1576>"
  Bus Selector11/7 -> Sensors_90/7(u7)  "<Value_1589>"
  Bus Selector11/8 -> Sensors_90/8(u8)  "<Value_1602>"
  Bus Selector11/9 -> Sensors_90/9(u9)  "<Value_1615>"
  Bus Selector11/10 -> Sensors_90/10(u10)  "<Value_1628>"
  Bus Selector11/11 -> Sensors_90/11(u11)  "<Value_1641>"
  Bus Selector11/12 -> Sensors_90/12(u12)  "<Value_1654>"
  Bus Selector11/13 -> Sensors_90/13(u13)  "<Value_1667>"
  Bus Selector11/14 -> Sensors_90/14(u14)  "<Value_1680>"
  Bus Selector11/15 -> Sensors_90/15(u15)  "<Value_1693>"
  OPC UA Handling 1/1 -> Bus Selector13/1, Bus Selector12/1, Bus Selector15/1, Bus Selector14/1
  Bus Selector12/1 -> AS-i_50/1(u1)  "<Value_1457>"
  Bus Selector12/2 -> AS-i_50/2(u2)  "<Value_1467>"
  Bus Selector12/3 -> AS-i_50/3(u3)  "<Value_1477>"
  Bus Selector12/4 -> AS-i_50/4(u4)  "<Value_1487>"
  Bus Selector12/5 -> AS-i_50/5(u5)  "<Value_1497>"
  Bus Selector12/6 -> AS-i_50/6(u6)  "<Value_1507>"
  Bus Selector12/7 -> AS-i_50/7(u7)  "<Value_1517>"
  Bus Selector12/8 -> AS-i_50/8(u8)  "<Value_1527>"
  Bus Selector12/9 -> AS-i_50/9(u9)  "<Value_1537>"
  Bus Selector12/10 -> AS-i_50/10(u10)  "<Value_1547>"
  Bus Selector12/11 -> AS-i_50/11(u11)  "<Value_1557>"
  Bus Selector12/12 -> AS-i_50/12(u12)  "<Value_1567>"
  Bus Selector13/1 -> Control_50/1(u1)  "<Value_1583>"
  Bus Selector13/2 -> Control_50/2(u2)  "<Value_1593>"
  Bus Selector13/3 -> Control_50/3(u3)  "<Value_1603>"
  Bus Selector13/4 -> Control_50/4(u4)  "<Value_1613>"
  Bus Selector13/5 -> Control_50/5(u5)  "<Value_1623>"
  Bus Selector14/1 -> Feedback_50/1(u1)  "<Value_1639>"
  Bus Selector14/2 -> Feedback_50/2(u2)  "<Value_1649>"
  Bus Selector14/3 -> Feedback_50/3(u3)  "<Value_1659>"
  Bus Selector14/4 -> Feedback_50/4(u4)  "<Value_1669>"
  Bus Selector14/5 -> Feedback_50/5(u5)  "<Value_1679>"
  Bus Selector14/6 -> Feedback_50/6(u6)  "<Value_1689>"
  Bus Selector14/7 -> Feedback_50/7(u7)  "<Value_1699>"
  Bus Selector14/8 -> Feedback_50/8(u8)  "<Value_1709>"
  Bus Selector14/9 -> Feedback_50/9(u9)  "<Value_1719>"
  Bus Selector14/10 -> Feedback_50/10(u10)  "<Value_1729>"
  Bus Selector14/11 -> Feedback_50/11(u11)  "<Value_1739>"
  Bus Selector14/12 -> Feedback_50/12(u12)  "<Value_1749>"
  Bus Selector15/1 -> Sensors_50/1(u1)  "<Value_1768>"
  Bus Selector15/2 -> Sensors_50/2(u2)  "<Value_1781>"
  Bus Selector15/3 -> Sensors_50/3(u3)  "<Value_1796>"
  Bus Selector15/4 -> Sensors_50/4(u4)  "<Value_1809>"
  Bus Selector15/5 -> Sensors_50/5(u5)  "<Value_1822>"
  Bus Selector15/6 -> Sensors_50/6(u6)  "<Value_1835>"
  Bus Selector15/7 -> Sensors_50/7(u7)  "<Value_1848>"
  Bus Selector15/8 -> Sensors_50/8(u8)  "<Value_1861>"
  Bus Selector15/9 -> Sensors_50/9(u9)  "<Value_1874>"
  Bus Selector15/10 -> Sensors_50/10(u10)  "<Value_1887>"
  Bus Selector15/11 -> Sensors_50/11(u11)  "<Value_1900>"
  Bus Selector15/12 -> Sensors_50/12(u12)  "<Value_1913>"
  Bus Selector15/13 -> Sensors_50/13(u13)  "<Value_1926>"
  Bus Selector15/14 -> Sensors_50/14(u14)  "<Value_1939>"
  Bus Selector15/15 -> Sensors_50/15(u15)  "<Value_1952>"
  OPC UA Distribution/1 -> Bus Selector17/1, Bus Selector18/1, Bus Selector16/1
  Bus Selector16/1 -> Control_80/1(u1)  "<Value_1195>"
  Bus Selector16/2 -> Control_80/2(u2)  "<Value_1205>"
  Bus Selector16/3 -> Control_80/3(u3)  "<Value_1215>"
  Bus Selector16/4 -> Control_80/4(u4)  "<Value_1227>"
  Bus Selector16/5 -> Control_80/5(u5)  "<Value_1239>"
  Bus Selector16/6 -> Control_80/6(u6)  "<Value_1249>"
  Bus Selector16/7 -> Control_80/7(u7)  "<Value_1261>"
  Bus Selector16/8 -> Control_80/8(u8)  "<Value_1271>"
  Bus Selector16/9 -> Control_80/9(u9)  "<Value_1281>"
  Bus Selector16/10 -> Control_80/10(u10)  "<Value_1291>"
  Bus Selector16/11 -> Control_80/11(u11)  "<Value_1301>"
  Bus Selector17/1 -> Feedback_80/1(u1)  "<Value_1317>"
  Bus Selector17/2 -> Feedback_80/2(u2)  "<Value_1327>"
  Bus Selector17/3 -> Feedback_80/3(u3)  "<Value_1337>"
  Bus Selector17/4 -> Feedback_80/4(u4)  "<Value_1347>"
  Bus Selector17/5 -> Feedback_80/5(u5)  "<Value_1357>"
  Bus Selector17/6 -> Feedback_80/6(u6)  "<Value_1367>"
  Bus Selector17/7 -> Feedback_80/7(u7)  "<Value_1377>"
  Bus Selector17/8 -> Feedback_80/8(u8)  "<Value_1387>"
  Bus Selector17/9 -> Feedback_80/9(u9)  "<Value_1397>"
  Bus Selector17/10 -> Feedback_80/10(u10)  "<Value_1407>"
  Bus Selector17/11 -> Feedback_80/11(u11)  "<Value_1417>"
  Bus Selector17/12 -> Feedback_80/12(u12)  "<Value_1427>"
  Bus Selector17/13 -> Feedback_80/13(u13)  "<Value_1437>"
  Bus Selector18/1 -> Sensors_80/1(u1)  "<Value_1458>"
  Bus Selector18/2 -> Sensors_80/2(u2)  "<Value_1471>"
  Bus Selector18/3 -> Sensors_80/3(u3)  "<Value_1486>"
  Bus Selector18/4 -> Sensors_80/4(u4)  "<Value_1499>"
  Bus Selector18/5 -> Sensors_80/5(u5)  "<Value_1512>"
  Bus Selector18/6 -> Sensors_80/6(u6)  "<Value_1525>"
  Bus Selector18/7 -> Sensors_80/7(u7)  "<Value_1538>"
  Bus Selector18/8 -> Sensors_80/8(u8)  "<Value_1551>"
  Bus Selector18/9 -> Sensors_80/9(u9)  "<Value_1564>"
  Bus Selector18/10 -> Sensors_80/10(u10)  "<Value_1577>"
  Bus Selector18/11 -> Sensors_80/11(u11)  "<Value_1590>"
  Bus Selector18/12 -> Sensors_80/12(u12)  "<Value_1603>"
  Bus Selector18/13 -> Sensors_80/13(u13)  "<Value_1616>"
  Bus Selector18/14 -> Sensors_80/14(u14)  "<Value_1629>"
  Bus Selector18/15 -> Sensors_80/15(u15)  "<Value_1642>"
  OPC UA Testing/1 -> Bus Selector21/1, Bus Selector22/1, Bus Selector20/1, Bus Selector19/1
  Bus Selector19/1 -> AS-i_70/1(u1)  "<Value_1455>"
  Bus Selector19/2 -> AS-i_70/2(u2)  "<Value_1465>"
  Bus Selector19/3 -> AS-i_70/3(u3)  "<Value_1475>"
  Bus Selector19/4 -> AS-i_70/4(u4)  "<Value_1485>"
  Bus Selector19/5 -> AS-i_70/5(u5)  "<Value_1495>"
  Bus Selector19/6 -> AS-i_70/6(u6)  "<Value_1505>"
  Bus Selector19/7 -> AS-i_70/7(u7)  "<Value_1515>"
  Bus Selector19/8 -> AS-i_70/8(u8)  "<Value_1525>"
  Bus Selector19/9 -> AS-i_70/9(u9)  "<Value_1535>"
  Bus Selector19/10 -> AS-i_70/10(u10)  "<Value_1545>"
  Bus Selector19/11 -> AS-i_70/11(u11)  "<Value_1555>"
  Bus Selector19/12 -> AS-i_70/12(u12)  "<Value_1565>"
  Bus Selector19/13 -> AS-i_70/13(u13)  "<Value_1575>"
  Bus Selector20/1 -> Control_70/1(u1)  "<Value_1591>"
  Bus Selector20/2 -> Control_70/2(u2)  "<Value_1601>"
  Bus Selector20/3 -> Control_70/3(u3)  "<Value_1611>"
  Bus Selector20/4 -> Control_70/4(u4)  "<Value_1621>"
  Bus Selector20/5 -> Control_70/5(u5)  "<Value_1631>"
  Bus Selector20/6 -> Control_70/6(u6)  "<Value_1641>"
  Bus Selector20/7 -> Control_70/7(u7)  "<Value_1651>"
  Bus Selector20/8 -> Control_70/8(u8)  "<Value_1661>"
  Bus Selector20/9 -> Control_70/9(u9)  "<Value_1671>"
  Bus Selector20/10 -> Control_70/10(u10)  "<Value_1681>"
  Bus Selector20/11 -> Control_70/11(u11)  "<Value_1691>"
  Bus Selector20/12 -> Control_70/12(u12)  "<Value_1701>"
  Bus Selector20/13 -> Control_70/13(u13)  "<Value_1711>"
  Bus Selector21/1 -> Feedback_70/1(u1)  "<Value_1727>"
  Bus Selector21/2 -> Feedback_70/2(u2)  "<Value_1737>"
  Bus Selector21/3 -> Feedback_70/3(u3)  "<Value_1747>"
  Bus Selector21/4 -> Feedback_70/4(u4)  "<Value_1757>"
  Bus Selector21/5 -> Feedback_70/5(u5)  "<Value_1767>"
  Bus Selector21/6 -> Feedback_70/6(u6)  "<Value_1777>"
  Bus Selector21/7 -> Feedback_70/7(u7)  "<Value_1787>"
  Bus Selector21/8 -> Feedback_70/8(u8)  "<Value_1797>"
  Bus Selector21/9 -> Feedback_70/9(u9)  "<Value_1807>"
  Bus Selector21/10 -> Feedback_70/10(u10)  "<Value_1817>"
  Bus Selector21/11 -> Feedback_70/11(u11)  "<Value_1827>"
  Bus Selector21/12 -> Feedback_70/12(u12)  "<Value_1837>"
  Bus Selector22/1 -> Sensors_70/1(u1)  "<Value_1858>"
  Bus Selector22/2 -> Sensors_70/2(u2)  "<Value_1871>"
  Bus Selector22/3 -> Sensors_70/3(u3)  "<Value_1886>"
  Bus Selector22/4 -> Sensors_70/4(u4)  "<Value_1899>"
  Bus Selector22/5 -> Sensors_70/5(u5)  "<Value_1912>"
  Bus Selector22/6 -> Sensors_70/6(u6)  "<Value_1925>"
  Bus Selector22/7 -> Sensors_70/7(u7)  "<Value_1938>"
  Bus Selector22/8 -> Sensors_70/8(u8)  "<Value_1951>"
  Bus Selector22/9 -> Sensors_70/9(u9)  "<Value_1964>"
  Bus Selector22/10 -> Sensors_70/10(u10)  "<Value_1977>"
  Bus Selector22/11 -> Sensors_70/11(u11)  "<Value_1990>"
  Bus Selector22/12 -> Sensors_70/12(u12)  "<Value_2003>"
  Bus Selector22/13 -> Sensors_70/13(u13)  "<Value_2016>"
  Bus Selector22/14 -> Sensors_70/14(u14)  "<Value_2029>"
  Bus Selector22/15 -> Sensors_70/15(u15)  "<Value_2042>"
  OPC UA Master/1 -> Bus Selector24/1, Bus Selector23/1, Bus Selector25/1
  Bus Selector23/1 -> Control_20/1(u1)  "<Value_1382>"
  Bus Selector23/2 -> Control_20/2(u2)  "<Value_1392>"
  Bus Selector23/3 -> Control_20/3(u3)  "<Value_1402>"
  Bus Selector23/4 -> Control_20/4(u4)  "<Value_1412>"
  Bus Selector23/5 -> Control_20/5(u5)  "<Value_1422>"
  Bus Selector23/6 -> Control_20/6(u6)  "<Value_1432>"
  Bus Selector23/7 -> Control_20/7(u7)  "<Value_1442>"
  Bus Selector23/8 -> Control_20/8(u8)  "<Value_1452>"
  Bus Selector23/9 -> Control_20/9(u9)  "<Value_1462>"
  Bus Selector23/10 -> Control_20/10(u10)  "<Value_1472>"
  Bus Selector23/11 -> Control_20/11(u11)  "<Value_1482>"
  Bus Selector23/12 -> Control_20/12(u12)  "<Value_1492>"
  Bus Selector23/13 -> Control_20/13(u13)  "<Value_1502>"
  Bus Selector23/14 -> Control_20/14(u14)  "<Value_1512>"
  Bus Selector23/15 -> Control_20/15(u15)  "<Value_1522>"
  Bus Selector23/16 -> Control_20/16(u16)  "<Value_1532>"
  Bus Selector23/17 -> Control_20/17(u17)  "<Value_1542>"
  Bus Selector23/18 -> Control_20/18(u18)  "<Value_1552>"
  Bus Selector23/19 -> Control_20/19(u19)  "<Value_1562>"
  Bus Selector23/20 -> Control_20/20(u20)  "<Value_1572>"
  Bus Selector23/21 -> Control_20/21(u21)  "<Value_1582>"
  Bus Selector23/22 -> Control_20/22(u22)  "<Value_1592>"
  Bus Selector23/23 -> Control_20/23(u23)  "<Value_1602>"
  Bus Selector23/24 -> Control_20/24(u24)  "<Value_1612>"
  Bus Selector24/1 -> Feedback_20/1(u1)  "<Value_1628>"
  Bus Selector24/2 -> Feedback_20/2(u2)  "<Value_1638>"
  Bus Selector24/3 -> Feedback_20/3(u3)  "<Value_1648>"
  Bus Selector24/4 -> Feedback_20/4(u4)  "<Value_1658>"
  Bus Selector24/5 -> Feedback_20/5(u5)  "<Value_1668>"
  Bus Selector24/6 -> Feedback_20/6(u6)  "<Value_1678>"
  Bus Selector24/7 -> Feedback_20/7(u7)  "<Value_1688>"
  Bus Selector24/8 -> Feedback_20/8(u8)  "<Value_1698>"
  Bus Selector24/9 -> Feedback_20/9(u9)  "<Value_1708>"
  Bus Selector25/1 -> Sensors_20/1(u1)  "<Value_1727>"
  Bus Selector25/2 -> Sensors_20/2(u2)  "<Value_1740>"
  Bus Selector25/3 -> Sensors_20/3(u3)  "<Value_1755>"
  Bus Selector25/4 -> Sensors_20/4(u4)  "<Value_1768>"
  Bus Selector25/5 -> Sensors_20/5(u5)  "<Value_1781>"
  Bus Selector25/6 -> Sensors_20/6(u6)  "<Value_1794>"
  Bus Selector25/7 -> Sensors_20/7(u7)  "<Value_1807>"
  Bus Selector25/8 -> Sensors_20/8(u8)  "<Value_1820>"
  Bus Selector25/9 -> Sensors_20/9(u9)  "<Value_1833>"
  Bus Selector25/10 -> Sensors_20/10(u10)  "<Value_1846>"
  Bus Selector25/11 -> Sensors_20/11(u11)  "<Value_1859>"
  Bus Selector25/12 -> Sensors_20/12(u12)  "<Value_1872>"
  Bus Selector25/13 -> Sensors_20/13(u13)  "<Value_1885>"
  Bus Selector25/14 -> Sensors_20/14(u14)  "<Value_1898>"
  Bus Selector25/15 -> Sensors_20/15(u15)  "<Value_1911>"
  Bus Selector25/16 -> Sensors_20/16(u16)  "<Value_1924>"
  Bus Selector25/17 -> Sensors_20/17(u17)  "<Value_1937>"
  Bus Selector25/18 -> Sensors_20/18(u18)  "<Value_1950>"
  Bus Selector25/19 -> Sensors_20/19(u19)  "<Value_1963>"
  Bus Selector25/20 -> Sensors_20/20(u20)  "<Value_1976>"
  Bus Selector25/21 -> Sensors_20/21(u21)  "<Value_1989>"
  Bus Selector25/22 -> Sensors_20/22(u22)  "<Value_2002>"
  Bus Selector25/23 -> Sensors_20/23(u23)  "<Value_2015>"
  Bus Selector25/24 -> Sensors_20/24(u24)  "<Value_2028>"
  Bus Selector25/25 -> Sensors_20/25(u25)  "<Value_2041>"
  Bus Selector25/26 -> Sensors_20/26(u26)  "<Value_2054>"
  Bus Selector25/27 -> Sensors_20/27(u27)  "<Value_2067>"
  Bus Selector25/28 -> Sensors_20/28(u28)  "<Value_2080>"
  Bus Selector25/29 -> Sensors_20/29(u29)  "<Value_2093>"
  Bus Selector25/30 -> Sensors_20/30(u30)  "<Value_2106>"
  Bus Selector25/31 -> Sensors_20/31(u31)  "<Value_2119>"
  Bus Selector25/32 -> Sensors_20/32(u32)  "<Value_2132>"
  Bus Selector25/33 -> Sensors_20/33(u33)  "<Value_2145>"
  OPC UA Processing/1 -> Bus Selector28/1, Bus Selector26/1, Bus Selector27/1
  Bus Selector26/1 -> Control_100/1(u1)  "<Value_1204>"
  Bus Selector26/2 -> Control_100/2(u2)  "<Value_1214>"
  Bus Selector26/3 -> Control_100/3(u3)  "<Value_1224>"
  Bus Selector26/4 -> Control_100/4(u4)  "<Value_1234>"
  Bus Selector26/5 -> Control_100/5(u5)  "<Value_1244>"
  Bus Selector26/6 -> Control_100/6(u6)  "<Value_1254>"
  Bus Selector26/7 -> Control_100/7(u7)  "<Value_1264>"
  Bus Selector26/8 -> Control_100/8(u8)  "<Value_1274>"
  Bus Selector26/9 -> Control_100/9(u9)  "<Value_1284>"
  Bus Selector26/10 -> Control_100/10(u10)  "<Value_1294>"
  Bus Selector27/1 -> Feedback_100/1(u1)  "<Value_1310>"
  Bus Selector27/2 -> Feedback_100/2(u2)  "<Value_1320>"
  Bus Selector27/3 -> Feedback_100/3(u3)  "<Value_1330>"
  Bus Selector27/4 -> Feedback_100/4(u4)  "<Value_1340>"
  Bus Selector27/5 -> Feedback_100/5(u5)  "<Value_1350>"
  Bus Selector27/6 -> Feedback_100/6(u6)  "<Value_1360>"
  Bus Selector27/7 -> Feedback_100/7(u7)  "<Value_1370>"
  Bus Selector27/8 -> Feedback_100/8(u8)  "<Value_1380>"
  Bus Selector27/9 -> Feedback_100/9(u9)  "<Value_1390>"
  Bus Selector27/10 -> Feedback_100/10(u10)  "<Value_1400>"
  Bus Selector27/11 -> Feedback_100/11(u11)  "<Value_1410>"
  Bus Selector27/12 -> Feedback_100/12(u12)  "<Value_1420>"
  Bus Selector27/13 -> Feedback_100/13(u13)  "<Value_1430>"
  Bus Selector27/14 -> Feedback_100/14(u14)  "<Value_1440>"
  Bus Selector28/1 -> Sensors_100/1(u1)  "<Value_1461>"
  Bus Selector28/2 -> Sensors_100/2(u2)  "<Value_1474>"
  Bus Selector28/3 -> Sensors_100/3(u3)  "<Value_1489>"
  Bus Selector28/4 -> Sensors_100/4(u4)  "<Value_1502>"
  Bus Selector28/5 -> Sensors_100/5(u5)  "<Value_1515>"
  Bus Selector28/6 -> Sensors_100/6(u6)  "<Value_1528>"
  Bus Selector28/7 -> Sensors_100/7(u7)  "<Value_1541>"
  Bus Selector28/8 -> Sensors_100/8(u8)  "<Value_1554>"
  Bus Selector28/9 -> Sensors_100/9(u9)  "<Value_1567>"
  Bus Selector28/10 -> Sensors_100/10(u10)  "<Value_1580>"
  Bus Selector28/11 -> Sensors_100/11(u11)  "<Value_1593>"
  Bus Selector28/12 -> Sensors_100/12(u12)  "<Value_1606>"
  Bus Selector28/13 -> Sensors_100/13(u13)  "<Value_1619>"
  Bus Selector28/14 -> Sensors_100/14(u14)  "<Value_1632>"
  Bus Selector28/15 -> Sensors_100/15(u15)  "<Value_1645>"
  OPC UA Sorting/1 -> Bus Selector31/1, Bus Selector30/1, Bus Selector29/1
  Bus Selector29/1 -> Control_60/1(u1)  "<Value_1178>"
  Bus Selector29/2 -> Control_60/2(u2)  "<Value_1188>"
  Bus Selector29/3 -> Control_60/3(u3)  "<Value_1198>"
  Bus Selector29/4 -> Control_60/4(u4)  "<Value_1208>"
  Bus Selector29/5 -> Control_60/5(u5)  "<Value_1218>"
  Bus Selector29/6 -> Control_60/6(u6)  "<Value_1228>"
  Bus Selector29/7 -> Control_60/7(u7)  "<Value_1238>"
  Bus Selector29/8 -> Control_60/8(u8)  "<Value_1248>"
  Bus Selector29/9 -> Control_60/9(u9)  "<Value_1258>"
  Bus Selector29/10 -> Control_60/10(u10)  "<Value_1268>"
  Bus Selector29/11 -> Control_60/11(u11)  "<Value_1278>"
  Bus Selector30/1 -> Feedback_60/1(u1)  "<Value_1294>"
  Bus Selector30/2 -> Feedback_60/2(u2)  "<Value_1304>"
  Bus Selector30/3 -> Feedback_60/3(u3)  "<Value_1314>"
  Bus Selector30/4 -> Feedback_60/4(u4)  "<Value_1324>"
  Bus Selector30/5 -> Feedback_60/5(u5)  "<Value_1334>"
  Bus Selector30/6 -> Feedback_60/6(u6)  "<Value_1344>"
  Bus Selector30/7 -> Feedback_60/7(u7)  "<Value_1354>"
  Bus Selector30/8 -> Feedback_60/8(u8)  "<Value_1364>"
  Bus Selector30/9 -> Feedback_60/9(u9)  "<Value_1374>"
  Bus Selector30/10 -> Feedback_60/10(u10)  "<Value_1384>"
  Bus Selector30/11 -> Feedback_60/11(u11)  "<Value_1394>"
  Bus Selector30/12 -> Feedback_60/12(u12)  "<Value_1404>"
  Bus Selector31/1 -> Sensors_60/1(u1)  "<Value_1423>"
  Bus Selector31/2 -> Sensors_60/2(u2)  "<Value_1436>"
  Bus Selector31/3 -> Sensors_60/3(u3)  "<Value_1451>"
  Bus Selector31/4 -> Sensors_60/4(u4)  "<Value_1464>"
  Bus Selector31/5 -> Sensors_60/5(u5)  "<Value_1477>"
  Bus Selector31/6 -> Sensors_60/6(u6)  "<Value_1490>"
  Bus Selector31/7 -> Sensors_60/7(u7)  "<Value_1503>"
  Bus Selector31/8 -> Sensors_60/8(u8)  "<Value_1516>"
  Bus Selector31/9 -> Sensors_60/9(u9)  "<Value_1529>"
  Bus Selector31/10 -> Sensors_60/10(u10)  "<Value_1542>"
  Bus Selector31/11 -> Sensors_60/11(u11)  "<Value_1555>"
  Bus Selector31/12 -> Sensors_60/12(u12)  "<Value_1568>"
  Bus Selector31/13 -> Sensors_60/13(u13)  "<Value_1581>"
  Bus Selector31/14 -> Sensors_60/14(u14)  "<Value_1594>"
  Bus Selector31/15 -> Sensors_60/15(u15)  "<Value_1607>"
  Bus Selector31/16 -> Sensors_60/16(u16)  "<Value_1620>"
  OPC UA Robot + Storage/1 -> Bus Selector5/1, Bus Selector4/1, Bus Selector6/1, Bus Selector7/1, Bus Selector3/1, Bus Selector2/1, Bus Selector1/1, Bus Selector/1
